simulink library "outp"  (R2021b)
(part 8 of 11)

      link override Signal_Override/_ovrdval: Value=KOUTP_FDCTHCREVentModeSta_enum_ovrdval
  VTHC_FDCTHCREVentYStaSet1_enum_Inproc : FVT_lib/outp/OverrideAndLimit  SystemSampleTime=-1  VariantActivationTime=update diagram  Latency=0  AutoFrameSizeCalculation=off
      link override Signal_Limit/_maxval: Value=KOUTP_FDCTHCREVentYStaSet1_enum_maxval
      link override Signal_Limit/_minval: Value=KOUTP_FDCTHCREVentYStaSet1_enum_minval
      link override Signal_Override/_ovrdflg: Value=KOUTP_FDCTHCREVentYStaSet1_enum_ovrdflg
      link override Signal_Override/_ovrdval: Value=KOUTP_FDCTHCREVentYStaSet1_enum_ovrdval
  VTHC_FDCTHCREVentYStaSet2_enum_Inproc : FVT_lib/outp/OverrideAndLimit  SystemSampleTime=-1  VariantActivationTime=update diagram  Latency=0  AutoFrameSizeCalculation=off
      link override Signal_Limit/_maxval: Value=KOUTP_FDCTHCREVentYStaSet2_enum_maxval
      link override Signal_Limit/_minval: Value=KOUTP_FDCTHCREVentYStaSet2_enum_minval
      link override Signal_Override/_ovrdflg: Value=KOUTP_FDCTHCREVentYStaSet2_enum_ovrdflg
      link override Signal_Override/_ovrdval: Value=KOUTP_FDCTHCREVentYStaSet2_enum_ovrdval
  VTHC_FDCTHCREVentYStaSet3_enum_Inproc : FVT_lib/outp/OverrideAndLimit  SystemSampleTime=-1  VariantActivationTime=update diagram  Latency=0  AutoFrameSizeCalculation=off
      link override Signal_Limit/_maxval: Value=KOUTP_FDCTHCREVentYStaSet3_enum_maxval
      link override Signal_Limit/_minval: Value=KOUTP_FDCTHCREVentYStaSet3_enum_minval
      link override Signal_Override/_ovrdflg: Value=KOUTP_FDCTHCREVentYStaSet3_enum_ovrdflg
      link override Signal_Override/_ovrdval: Value=KOUTP_FDCTHCREVentYStaSet3_enum_ovrdval
  VTHC_FDCTHCREVentYStaSet4_enum_Inproc : FVT_lib/outp/OverrideAndLimit  SystemSampleTime=-1  VariantActivationTime=update diagram  Latency=0  AutoFrameSizeCalculation=off
      link override Signal_Limit/_maxval: Value=KOUTP_FDCTHCREVentYStaSet4_enum_maxval
      link override Signal_Limit/_minval: Value=KOUTP_FDCTHCREVentYStaSet4_enum_minval
      link override Signal_Override/_ovrdflg: Value=KOUTP_FDCTHCREVentYStaSet4_enum_ovrdflg
      link override Signal_Override/_ovrdval: Value=KOUTP_FDCTHCREVentYStaSet4_enum_ovrdval
  VTHC_FDCTHCREVentYStaSet5_enum_Inproc : FVT_lib/outp/OverrideAndLimit  SystemSampleTime=-1  VariantActivationTime=update diagram  Latency=0  AutoFrameSizeCalculation=off
      link override Signal_Limit/_maxval: Value=KOUTP_FDCTHCREVentYStaSet5_enum_maxval
      link override Signal_Limit/_minval: Value=KOUTP_FDCTHCREVentYStaSet5_enum_minval
      link override Signal_Override/_ovrdflg: Value=KOUTP_FDCTHCREVentYStaSet5_enum_ovrdflg
      link override Signal_Override/_ovrdval: Value=KOUTP_FDCTHCREVentYStaSet5_enum_ovrdval
  VTHC_FDCTHCREVentYStaSet7_enum_Inproc : FVT_lib/outp/OverrideAndLimit  SystemSampleTime=-1  VariantActivationTime=update diagram  Latency=0  AutoFrameSizeCalculation=off
      link override Signal_Limit/_maxval: Value=KOUTP_FDCTHCREVentYStaSet7_enum_maxval
      link override Signal_Limit/_minval: Value=KOUTP_FDCTHCREVentYStaSet7_enum_minval
      link override Signal_Override/_ovrdflg: Value=KOUTP_FDCTHCREVentYStaSet7_enum_ovrdflg
      link override Signal_Override/_ovrdval: Value=KOUTP_FDCTHCREVentYStaSet7_enum_ovrdval
  VTHC_FDCTHCREVentYSta_enum_Inproc : FVT_lib/outp/OverrideAndLimit  SystemSampleTime=-1  VariantActivationTime=update diagram  Latency=0  AutoFrameSizeCalculation=off
      link override Signal_Limit/_maxval: Value=KOUTP_FDCTHCREVentYSta_enum_maxval
      link override Signal_Limit/_minval: Value=KOUTP_FDCTHCREVentYSta_enum_minval
      link override Signal_Override/_ovrdflg: Value=KOUTP_FDCTHCREVentYSta_enum_ovrdflg
      link override Signal_Override/_ovrdval: Value=KOUTP_FDCTHCREVentYSta_enum_ovrdval
  VTHC_FDCTHCREVentZStaSet1_enum_Inproc : FVT_lib/outp/OverrideAndLimit  SystemSampleTime=-1  VariantActivationTime=update diagram  Latency=0  AutoFrameSizeCalculation=off
      link override Signal_Limit/_maxval: Value=KOUTP_FDCTHCREVentZStaSet1_enum_maxval
      link override Signal_Limit/_minval: Value=KOUTP_FDCTHCREVentZStaSet1_enum_minval
      link override Signal_Override/_ovrdflg: Value=KOUTP_FDCTHCREVentZStaSet1_enum_ovrdflg
      link override Signal_Override/_ovrdval: Value=KOUTP_FDCTHCREVentZStaSet1_enum_ovrdval
  VTHC_FDCTHCREVentZStaSet2_enum_Inproc : FVT_lib/outp/OverrideAndLimit  SystemSampleTime=-1  VariantActivationTime=update diagram  Latency=0  AutoFrameSizeCalculation=off
      link override Signal_Limit/_maxval: Value=KOUTP_FDCTHCREVentZStaSet2_enum_maxval
      link override Signal_Limit/_minval: Value=KOUTP_FDCTHCREVentZStaSet2_enum_minval
      link override Signal_Override/_ovrdflg: Value=KOUTP_FDCTHCREVentZStaSet2_enum_ovrdflg
      link override Signal_Override/_ovrdval: Value=KOUTP_FDCTHCREVentZStaSet2_enum_ovrdval
  VTHC_FDCTHCREVentZStaSet3_enum_Inproc : FVT_lib/outp/OverrideAndLimit  SystemSampleTime=-1  VariantActivationTime=update diagram  Latency=0  AutoFrameSizeCalculation=off
      link override Signal_Limit/_maxval: Value=KOUTP_FDCTHCREVentZStaSet3_enum_maxval
      link override Signal_Limit/_minval: Value=KOUTP_FDCTHCREVentZStaSet3_enum_minval
      link override Signal_Override/_ovrdflg: Value=KOUTP_FDCTHCREVentZStaSet3_enum_ovrdflg
      link override Signal_Override/_ovrdval: Value=KOUTP_FDCTHCREVentZStaSet3_enum_ovrdval
  VTHC_FDCTHCREVentZStaSet4_enum_Inproc : FVT_lib/outp/OverrideAndLimit  SystemSampleTime=-1  VariantActivationTime=update diagram  Latency=0  AutoFrameSizeCalculation=off
      link override Signal_Limit/_maxval: Value=KOUTP_FDCTHCREVentZStaSet4_enum_maxval
      link override Signal_Limit/_minval: Value=KOUTP_FDCTHCREVentZStaSet4_enum_minval
      link override Signal_Override/_ovrdflg: Value=KOUTP_FDCTHCREVentZStaSet4_enum_ovrdflg
      link override Signal_Override/_ovrdval: Value=KOUTP_FDCTHCREVentZStaSet4_enum_ovrdval
  VTHC_FDCTHCREVentZStaSet5_enum_Inproc : FVT_lib/outp/OverrideAndLimit  SystemSampleTime=-1  VariantActivationTime=update diagram  Latency=0  AutoFrameSizeCalculation=off
      link override Signal_Limit/_maxval: Value=KOUTP_FDCTHCREVentZStaSet5_enum_maxval
      link override Signal_Limit/_minval: Value=KOUTP_FDCTHCREVentZStaSet5_enum_minval
      link override Signal_Override/_ovrdflg: Value=KOUTP_FDCTHCREVentZStaSet5_enum_ovrdflg
      link override Signal_Override/_ovrdval: Value=KOUTP_FDCTHCREVentZStaSet5_enum_ovrdval
  VTHC_FDCTHCREVentZStaSet7_enum_Inproc : FVT_lib/outp/OverrideAndLimit  SystemSampleTime=-1  VariantActivationTime=update diagram  Latency=0  AutoFrameSizeCalculation=off
      link override Signal_Limit/_maxval: Value=KOUTP_FDCTHCREVentZStaSet7_enum_maxval
      link override Signal_Limit/_minval: Value=KOUTP_FDCTHCREVentZStaSet7_enum_minval
      link override Signal_Override/_ovrdflg: Value=KOUTP_FDCTHCREVentZStaSet7_enum_ovrdflg
      link override Signal_Override/_ovrdval: Value=KOUTP_FDCTHCREVentZStaSet7_enum_ovrdval
  VTHC_FDCTHCREVentZSta_enum_Inproc : FVT_lib/outp/OverrideAndLimit  SystemSampleTime=-1  VariantActivationTime=update diagram  Latency=0  AutoFrameSizeCalculation=off
      link override Signal_Limit/_maxval: Value=KOUTP_FDCTHCREVentZSta_enum_maxval
      link override Signal_Limit/_minval: Value=KOUTP_FDCTHCREVentZSta_enum_minval
      link override Signal_Override/_ovrdflg: Value=KOUTP_FDCTHCREVentZSta_enum_ovrdflg
      link override Signal_Override/_ovrdval: Value=KOUTP_FDCTHCREVentZSta_enum_ovrdval
  VTHC_FDCTHCRVentENSta_flg_Inproc : FVT_lib/outp/OverrideAndLimit  SystemSampleTime=-1  VariantActivationTime=update diagram  Latency=0  AutoFrameSizeCalculation=off
      link override Signal_Limit/_maxval: Value=KOUTP_FDCTHCRVentENSta_flg_maxval
      link override Signal_Limit/_minval: Value=KOUTP_FDCTHCRVentENSta_flg_minval
      link override Signal_Override/_ovrdflg: Value=KOUTP_FDCTHCRVentENSta_flg_ovrdflg
      link override Signal_Override/_ovrdval: Value=KOUTP_FDCTHCRVentENSta_flg_ovrdval
  VTHC_FDCompCmd_rpm_Inproc : FVT_lib/outp/OverrideAndLimit  SystemSampleTime=-1  VariantActivationTime=update diagram  Latency=0  AutoFrameSizeCalculation=off
      link override Signal_Limit/_maxval: Value=KOUTP_FDCompCmd_rpm_maxval
      link override Signal_Limit/_minval: Value=KOUTP_FDCompCmd_rpm_minval
      link override Signal_Override/_ovrdflg: Value=KOUTP_FDCompCmd_rpm_ovrdflg
      link override Signal_Override/_ovrdval: Value=KOUTP_FDCompCmd_rpm_ovrdval
  VTHC_FDEWP1Cmd_enum_Inproc : FVT_lib/outp/OverrideAndLimit  SystemSampleTime=-1  VariantActivationTime=update diagram  Latency=0  AutoFrameSizeCalculation=off
      link override Signal_Limit/_maxval: Value=KOUTP_FDEWP1Cmd_enum_maxval
      link override Signal_Limit/_minval: Value=KOUTP_FDEWP1Cmd_enum_minval
      link override Signal_Override/_ovrdflg: Value=KOUTP_FDEWP1Cmd_enum_ovrdflg
      link override Signal_Override/_ovrdval: Value=KOUTP_FDEWP1Cmd_enum_ovrdval
  VTHC_FDEWP2Cmd_enum_Inproc : FVT_lib/outp/OverrideAndLimit  SystemSampleTime=-1  VariantActivationTime=update diagram  Latency=0  AutoFrameSizeCalculation=off
      link override Signal_Limit/_maxval: Value=KOUTP_FDEWP2Cmd_enum_maxval
      link override Signal_Limit/_minval: Value=KOUTP_FDEWP2Cmd_enum_minval
      link override Signal_Override/_ovrdflg: Value=KOUTP_FDEWP2Cmd_enum_ovrdflg
      link override Signal_Override/_ovrdval: Value=KOUTP_FDEWP2Cmd_enum_ovrdval
  VTHC_FDEWP3Cmd_enum_Inproc : FVT_lib/outp/OverrideAndLimit  SystemSampleTime=-1  VariantActivationTime=update diagram  Latency=0  AutoFrameSizeCalculation=off
      link override Signal_Limit/_maxval: Value=KOUTP_FDEWP3Cmd_enum_maxval
      link override Signal_Limit/_minval: Value=KOUTP_FDEWP3Cmd_enum_minval
      link override Signal_Override/_ovrdflg: Value=KOUTP_FDEWP3Cmd_enum_ovrdflg
      link override Signal_Override/_ovrdval: Value=KOUTP_FDEWP3Cmd_enum_ovrdval
  VTHC_FDEXV1Cmd_step_Inproc : FVT_lib/outp/OverrideAndLimit  SystemSampleTime=-1  VariantActivationTime=update diagram  Latency=0  AutoFrameSizeCalculation=off
      link override Signal_Limit/_maxval: Value=KOUTP_FDEXV1Cmd_step_maxval
      link override Signal_Limit/_minval: Value=KOUTP_FDEXV1Cmd_step_minval
      link override Signal_Override/_ovrdflg: Value=KOUTP_FDEXV1Cmd_step_ovrdflg
      link override Signal_Override/_ovrdval: Value=KOUTP_FDEXV1Cmd_step_ovrdval
  VTHC_FDEXV2Cmd_step_Inproc : FVT_lib/outp/OverrideAndLimit  SystemSampleTime=-1  VariantActivationTime=update diagram  Latency=0  AutoFrameSizeCalculation=off
      link override Signal_Limit/_maxval: Value=KOUTP_FDEXV2Cmd_step_maxval
      link override Signal_Limit/_minval: Value=KOUTP_FDEXV2Cmd_step_minval
      link override Signal_Override/_ovrdflg: Value=KOUTP_FDEXV2Cmd_step_ovrdflg
      link override Signal_Override/_ovrdval: Value=KOUTP_FDEXV2Cmd_step_ovrdval
  VTHC_FDFWVCmd_flg_Inproc : FVT_lib/outp/OverrideAndLimit  SystemSampleTime=-1  VariantActivationTime=update diagram  Latency=0  AutoFrameSizeCalculation=off
      link override Signal_Limit/_maxval: Value=KOUTP_FDFWVCmd_flg_maxval
      link override Signal_Limit/_minval: Value=KOUTP_FDFWVCmd_flg_minval
      link override Signal_Override/_ovrdflg: Value=KOUTP_FDFWVCmd_flg_ovrdflg
      link override Signal_Override/_ovrdval: Value=KOUTP_FDFWVCmd_flg_ovrdval
  VTHC_FDFrLeAPTCHeatPwrCmd_W_Inproc : FVT_lib/outp/OverrideAndLimit  SystemSampleTime=-1  VariantActivationTime=update diagram  Latency=0  AutoFrameSizeCalculation=off
      link override Signal_Limit/_maxval: Value=KOUTP_FDFrLeAPTCHeatPwrCmd_W_maxval
      link override Signal_Limit/_minval: Value=KOUTP_FDFrLeAPTCHeatPwrCmd_W_minval
      link override Signal_Override/_ovrdflg: Value=KOUTP_FDFrLeAPTCHeatPwrCmd_W_ovrdflg
      link override Signal_Override/_ovrdval: Value=KOUTP_FDFrLeAPTCHeatPwrCmd_W_ovrdval
  VTHC_FDFrRiAPTCHeatPwrCmd_W_Inproc : FVT_lib/outp/OverrideAndLimit  SystemSampleTime=-1  VariantActivationTime=update diagram  Latency=0  AutoFrameSizeCalculation=off
      link override Signal_Limit/_maxval: Value=KOUTP_FDFrRiAPTCHeatPwrCmd_W_maxval
      link override Signal_Limit/_minval: Value=KOUTP_FDFrRiAPTCHeatPwrCmd_W_minval
      link override Signal_Override/_ovrdflg: Value=KOUTP_FDFrRiAPTCHeatPwrCmd_W_ovrdflg
      link override Signal_Override/_ovrdval: Value=KOUTP_FDFrRiAPTCHeatPwrCmd_W_ovrdval
  VTHC_FDFrWPTCHeatPwrCmd_W_Inproc : FVT_lib/outp/OverrideAndLimit  SystemSampleTime=-1  VariantActivationTime=update diagram  Latency=0  AutoFrameSizeCalculation=off
      link override Signal_Limit/_maxval: Value=KOUTP_FDFrWPTCHeatPwrCmd_W_maxval
      link override Signal_Limit/_minval: Value=KOUTP_FDFrWPTCHeatPwrCmd_W_minval
      link override Signal_Override/_ovrdflg: Value=KOUTP_FDFrWPTCHeatPwrCmd_W_ovrdflg
      link override Signal_Override/_ovrdval: Value=KOUTP_FDFrWPTCHeatPwrCmd_W_ovrdval
  VTHC_FDRecyAutoCmd_enum_Inproc : FVT_lib/outp/OverrideAndLimit  SystemSampleTime=-1  VariantActivationTime=update diagram  Latency=0  AutoFrameSizeCalculation=off
      link override Signal_Limit/_maxval: Value=KOUTP_FDRecyAutoCmd_enum_maxval
      link override Signal_Limit/_minval: Value=KOUTP_FDRecyAutoCmd_enum_minval
      link override Signal_Override/_ovrdflg: Value=KOUTP_FDRecyAutoCmd_enum_ovrdflg
      link override Signal_Override/_ovrdval: Value=KOUTP_FDRecyAutoCmd_enum_ovrdval
  VTHC_FDRrAPTCHeatPwrCmd_W_Inproc : FVT_lib/outp/OverrideAndLimit  SystemSampleTime=-1  VariantActivationTime=update diagram  Latency=0  AutoFrameSizeCalculation=off
      link override Signal_Limit/_maxval: Value=KOUTP_FDRrAPTCHeatPwrCmd_W_maxval
      link override Signal_Limit/_minval: Value=KOUTP_FDRrAPTCHeatPwrCmd_W_minval
      link override Signal_Override/_ovrdflg: Value=KOUTP_FDRrAPTCHeatPwrCmd_W_ovrdflg
      link override Signal_Override/_ovrdval: Value=KOUTP_FDRrAPTCHeatPwrCmd_W_ovrdval
  VTHC_FDSOTXVCmd_flg_Inproc : FVT_lib/outp/OverrideAndLimit  SystemSampleTime=-1  VariantActivationTime=update diagram  Latency=0  AutoFrameSizeCalculation=off
      link override Signal_Limit/_maxval: Value=KOUTP_FDSOTXVCmd_flg_maxval
      link override Signal_Limit/_minval: Value=KOUTP_FDSOTXVCmd_flg_minval
      link override Signal_Override/_ovrdflg: Value=KOUTP_FDSOTXVCmd_flg_ovrdflg
      link override Signal_Override/_ovrdval: Value=KOUTP_FDSOTXVCmd_flg_ovrdval
  VTHC_FDSOV1Cmd_flg_Inproc : FVT_lib/outp/OverrideAndLimit  SystemSampleTime=-1  VariantActivationTime=update diagram  Latency=0  AutoFrameSizeCalculation=off
      link override Signal_Limit/_maxval: Value=KOUTP_FDSOV1Cmd_flg_maxval
      link override Signal_Limit/_minval: Value=KOUTP_FDSOV1Cmd_flg_minval
      link override Signal_Override/_ovrdflg: Value=KOUTP_FDSOV1Cmd_flg_ovrdflg
      link override Signal_Override/_ovrdval: Value=KOUTP_FDSOV1Cmd_flg_ovrdval
  VTHC_FDSOV2Cmd_flg_Inproc : FVT_lib/outp/OverrideAndLimit  SystemSampleTime=-1  VariantActivationTime=update diagram  Latency=0  AutoFrameSizeCalculation=off
      link override Signal_Limit/_maxval: Value=KOUTP_FDSOV2Cmd_flg_maxval
      link override Signal_Limit/_minval: Value=KOUTP_FDSOV2Cmd_flg_minval
      link override Signal_Override/_ovrdflg: Value=KOUTP_FDSOV2Cmd_flg_ovrdflg
      link override Signal_Override/_ovrdval: Value=KOUTP_FDSOV2Cmd_flg_ovrdval
  VTHC_FDSOV3Cmd_flg_Inproc : FVT_lib/outp/OverrideAndLimit  SystemSampleTime=-1  VariantActivationTime=update diagram  Latency=0  AutoFrameSizeCalculation=off
      link override Signal_Limit/_maxval: Value=KOUTP_FDSOV3Cmd_flg_maxval
      link override Signal_Limit/_minval: Value=KOUTP_FDSOV3Cmd_flg_minval
      link override Signal_Override/_ovrdflg: Value=KOUTP_FDSOV3Cmd_flg_ovrdflg
      link override Signal_Override/_ovrdval: Value=KOUTP_FDSOV3Cmd_flg_ovrdval
  VTHC_FDTWVCmd_pct_Inproc : FVT_lib/outp/OverrideAndLimit  SystemSampleTime=-1  VariantActivationTime=update diagram  Latency=0  AutoFrameSizeCalculation=off
      link override Signal_Limit/_maxval: Value=KOUTP_FDTWVCmd_pct_maxval
      link override Signal_Limit/_minval: Value=KOUTP_FDTWVCmd_pct_minval
      link override Signal_Override/_ovrdflg: Value=KOUTP_FDTWVCmd_pct_ovrdflg
      link override Signal_Override/_ovrdval: Value=KOUTP_FDTWVCmd_pct_ovrdval
  VTHC_FOOTSet_enum_Inproc : FVT_lib/outp/OverrideAndLimit  SystemSampleTime=-1  VariantActivationTime=update diagram  Latency=0  AutoFrameSizeCalculation=off
      link override Signal_Limit/_maxval: Value=KOUTP_FOOTSet_enum_maxval
      link override Signal_Limit/_minval: Value=KOUTP_FOOTSet_enum_minval
      link override Signal_Override/_ovrdflg: Value=KOUTP_FOOTSet_enum_ovrdflg
      link override Signal_Override/_ovrdval: Value=KOUTP_FOOTSet_enum_ovrdval
  VTHC_FaceMSet_enum_Inproc : FVT_lib/outp/OverrideAndLimit  SystemSampleTime=-1  VariantActivationTime=update diagram  Latency=0  AutoFrameSizeCalculation=off
      link override Signal_Limit/_maxval: Value=KOUTP_FaceMSet_enum_maxval
      link override Signal_Limit/_minval: Value=KOUTP_FaceMSet_enum_minval
      link override Signal_Override/_ovrdflg: Value=KOUTP_FaceMSet_enum_ovrdflg
      link override Signal_Override/_ovrdval: Value=KOUTP_FaceMSet_enum_ovrdval
  VTHC_FaceM_flg_Inproc : FVT_lib/outp/OverrideAndLimit  SystemSampleTime=-1  VariantActivationTime=update diagram  Latency=0  AutoFrameSizeCalculation=off
      link override Signal_Limit/_maxval: Value=KOUTP_FaceM_flg_maxval
      link override Signal_Limit/_minval: Value=KOUTP_FaceM_flg_minval
      link override Signal_Override/_ovrdflg: Value=KOUTP_FaceM_flg_ovrdflg
      link override Signal_Override/_ovrdval: Value=KOUTP_FaceM_flg_ovrdval
  VTHC_Face_flg_Inproc : FVT_lib/outp/OverrideAndLimit  SystemSampleTime=-1  VariantActivationTime=update diagram  Latency=0  AutoFrameSizeCalculation=off
      link override Signal_Limit/_maxval: Value=KOUTP_Face_flg_maxval
      link override Signal_Limit/_minval: Value=KOUTP_Face_flg_minval
      link override Signal_Override/_ovrdflg: Value=KOUTP_Face_flg_ovrdflg
      link override Signal_Override/_ovrdval: Value=KOUTP_Face_flg_ovrdval
  VTHC_FootMSet_enum_Inproc : FVT_lib/outp/OverrideAndLimit  SystemSampleTime=-1  VariantActivationTime=update diagram  Latency=0  AutoFrameSizeCalculation=off
      link override Signal_Limit/_maxval: Value=KOUTP_FootMSet_enum_maxval
      link override Signal_Limit/_minval: Value=KOUTP_FootMSet_enum_minval
      link override Signal_Override/_ovrdflg: Value=KOUTP_FootMSet_enum_ovrdflg
      link override Signal_Override/_ovrdval: Value=KOUTP_FootMSet_enum_ovrdval
  VTHC_FootM_flg_Inproc : FVT_lib/outp/OverrideAndLimit  SystemSampleTime=-1  VariantActivationTime=update diagram  Latency=0  AutoFrameSizeCalculation=off
      link override Signal_Limit/_maxval: Value=KOUTP_FootM_flg_maxval
      link override Signal_Limit/_minval: Value=KOUTP_FootM_flg_minval
      link override Signal_Override/_ovrdflg: Value=KOUTP_FootM_flg_ovrdflg
      link override Signal_Override/_ovrdval: Value=KOUTP_FootM_flg_ovrdval
  VTHC_Foot_flg_Inproc : FVT_lib/outp/OverrideAndLimit  SystemSampleTime=-1  VariantActivationTime=update diagram  Latency=0  AutoFrameSizeCalculation=off
      link override Signal_Limit/_maxval: Value=KOUTP_Foot_flg_maxval
      link override Signal_Limit/_minval: Value=KOUTP_Foot_flg_minval
      link override Signal_Override/_ovrdflg: Value=KOUTP_Foot_flg_ovrdflg
      link override Signal_Override/_ovrdval: Value=KOUTP_Foot_flg_ovrdval
  VTHC_FrostSet_enum_Inproc : FVT_lib/outp/OverrideAndLimit  SystemSampleTime=-1  VariantActivationTime=update diagram  Latency=0  AutoFrameSizeCalculation=off
      link override Signal_Limit/_maxval: Value=KOUTP_FrostSet_enum_maxval
      link override Signal_Limit/_minval: Value=KOUTP_FrostSet_enum_minval
      link override Signal_Override/_ovrdflg: Value=KOUTP_FrostSet_enum_ovrdflg
      link override Signal_Override/_ovrdval: Value=KOUTP_FrostSet_enum_ovrdval
  VTHC_Frost_flg_Inproc : FVT_lib/outp/OverrideAndLimit  SystemSampleTime=-1  VariantActivationTime=update diagram  Latency=0  AutoFrameSizeCalculation=off
      link override Signal_Limit/_maxval: Value=KOUTP_Frost_flg_maxval
      link override Signal_Limit/_minval: Value=KOUTP_Frost_flg_minval
      link override Signal_Override/_ovrdflg: Value=KOUTP_Frost_flg_ovrdflg
      link override Signal_Override/_ovrdval: Value=KOUTP_Frost_flg_ovrdval
  VTHC_IONSWStaSet_enum_Inproc : FVT_lib/outp/OverrideAndLimit  SystemSampleTime=-1  VariantActivationTime=update diagram  Latency=0  AutoFrameSizeCalculation=off
      link override Signal_Limit/_maxval: Value=KOUTP_IONSWStaSet_enum_maxval
      link override Signal_Limit/_minval: Value=KOUTP_IONSWStaSet_enum_minval
      link override Signal_Override/_ovrdflg: Value=KOUTP_IONSWStaSet_enum_ovrdflg
      link override Signal_Override/_ovrdval: Value=KOUTP_IONSWStaSet_enum_ovrdval
  VTHC_LEVentModeStaSet123_enum_Inproc : FVT_lib/outp/OverrideAndLimit  SystemSampleTime=-1  VariantActivationTime=update diagram  Latency=0  AutoFrameSizeCalculation=off
      link override Signal_Limit/_maxval: Value=KOUTP_LEVentModeStaSet123_enum_maxval
      link override Signal_Limit/_minval: Value=KOUTP_LEVentModeStaSet123_enum_minval
      link override Signal_Override/_ovrdflg: Value=KOUTP_LEVentModeStaSet123_enum_ovrdflg
      link override Signal_Override/_ovrdval: Value=KOUTP_LEVentModeStaSet123_enum_ovrdval
  VTHC_LEVentModeStaSet457_enum_Inproc : FVT_lib/outp/OverrideAndLimit  SystemSampleTime=-1  VariantActivationTime=update diagram  Latency=0  AutoFrameSizeCalculation=off
      link override Signal_Limit/_maxval: Value=KOUTP_LEVentModeStaSet457_enum_maxval
      link override Signal_Limit/_minval: Value=KOUTP_LEVentModeStaSet457_enum_minval
      link override Signal_Override/_ovrdflg: Value=KOUTP_LEVentModeStaSet457_enum_ovrdflg
      link override Signal_Override/_ovrdval: Value=KOUTP_LEVentModeStaSet457_enum_ovrdval
  VTHC_LVentENSet_enum_Inproc : FVT_lib/outp/OverrideAndLimit  SystemSampleTime=-1  VariantActivationTime=update diagram  Latency=0  AutoFrameSizeCalculation=off
      link override Signal_Limit/_maxval: Value=KOUTP_LVentENSet_enum_maxval
      link override Signal_Limit/_minval: Value=KOUTP_LVentENSet_enum_minval
      link override Signal_Override/_ovrdflg: Value=KOUTP_LVentENSet_enum_ovrdflg
      link override Signal_Override/_ovrdval: Value=KOUTP_LVentENSet_enum_ovrdval
  VTHC_LVentEN_flg_Inproc : FVT_lib/outp/OverrideAndLimit  SystemSampleTime=-1  VariantActivationTime=update diagram  Latency=0  AutoFrameSizeCalculation=off
      link override Signal_Limit/_maxval: Value=KOUTP_LVentEN_flg_maxval
      link override Signal_Limit/_minval: Value=KOUTP_LVentEN_flg_minval
      link override Signal_Override/_ovrdflg: Value=KOUTP_LVentEN_flg_ovrdflg
      link override Signal_Override/_ovrdval: Value=KOUTP_LVentEN_flg_ovrdval
  VTHC_REVentModeStaSet123_enum_Inproc : FVT_lib/outp/OverrideAndLimit  SystemSampleTime=-1  VariantActivationTime=update diagram  Latency=0  AutoFrameSizeCalculation=off
      link override Signal_Limit/_maxval: Value=KOUTP_REVentModeStaSet123_enum_maxval
      link override Signal_Limit/_minval: Value=KOUTP_REVentModeStaSet123_enum_minval
      link override Signal_Override/_ovrdflg: Value=KOUTP_REVentModeStaSet123_enum_ovrdflg
      link override Signal_Override/_ovrdval: Value=KOUTP_REVentModeStaSet123_enum_ovrdval
  VTHC_REVentModeStaSet457_enum_Inproc : FVT_lib/outp/OverrideAndLimit  SystemSampleTime=-1  VariantActivationTime=update diagram  Latency=0  AutoFrameSizeCalculation=off
      link override Signal_Limit/_maxval: Value=KOUTP_REVentModeStaSet457_enum_maxval
      link override Signal_Limit/_minval: Value=KOUTP_REVentModeStaSet457_enum_minval
      link override Signal_Override/_ovrdflg: Value=KOUTP_REVentModeStaSet457_enum_ovrdflg
      link override Signal_Override/_ovrdval: Value=KOUTP_REVentModeStaSet457_enum_ovrdval
  VTHC_RVentENSet_enum_Inproc : FVT_lib/outp/OverrideAndLimit  SystemSampleTime=-1  VariantActivationTime=update diagram  Latency=0  AutoFrameSizeCalculation=off
      link override Signal_Limit/_maxval: Value=KOUTP_RVentENSet_enum_maxval
      link override Signal_Limit/_minval: Value=KOUTP_RVentENSet_enum_minval
      link override Signal_Override/_ovrdflg: Value=KOUTP_RVentENSet_enum_ovrdflg
      link override Signal_Override/_ovrdval: Value=KOUTP_RVentENSet_enum_ovrdval
  VTHC_RVentEN_flg_Inproc : FVT_lib/outp/OverrideAndLimit  SystemSampleTime=-1  VariantActivationTime=update diagram  Latency=0  AutoFrameSizeCalculation=off
      link override Signal_Limit/_maxval: Value=KOUTP_RVentEN_flg_maxval
      link override Signal_Limit/_minval: Value=KOUTP_RVentEN_flg_minval
      link override Signal_Override/_ovrdflg: Value=KOUTP_RVentEN_flg_ovrdflg
      link override Signal_Override/_ovrdval: Value=KOUTP_RVentEN_flg_ovrdval
  VTHC_RecAutoFlg_flg_Inproc : FVT_lib/outp/OverrideAndLimit  SystemSampleTime=-1  VariantActivationTime=update diagram  Latency=0  AutoFrameSizeCalculation=off
      link override Signal_Limit/_maxval: Value=KOUTP_RecAutoFlg_flg_maxval
      link override Signal_Limit/_minval: Value=KOUTP_RecAutoFlg_flg_minval
      link override Signal_Override/_ovrdflg: Value=KOUTP_RecAutoFlg_flg_ovrdflg
      link override Signal_Override/_ovrdval: Value=KOUTP_RecAutoFlg_flg_ovrdval
  VTHC_RecyAutoSet_enum_Inproc : FVT_lib/outp/OverrideAndLimit  SystemSampleTime=-1  VariantActivationTime=update diagram  Latency=0  AutoFrameSizeCalculation=off
      link override Signal_Limit/_maxval: Value=KOUTP_RecyAutoSet_enum_maxval
      link override Signal_Limit/_minval: Value=KOUTP_RecyAutoSet_enum_minval
      link override Signal_Override/_ovrdflg: Value=KOUTP_RecyAutoSet_enum_ovrdflg
      link override Signal_Override/_ovrdval: Value=KOUTP_RecyAutoSet_enum_ovrdval
  VTHC_SettempZon1Set1_enum_Inproc : FVT_lib/outp/OverrideAndLimit  SystemSampleTime=-1  VariantActivationTime=update diagram  Latency=0  AutoFrameSizeCalculation=off
      link override Signal_Limit/_maxval: Value=KOUTP_SettempZon1Set1_enum_maxval
      link override Signal_Limit/_minval: Value=KOUTP_SettempZon1Set1_enum_minval
      link override Signal_Override/_ovrdflg: Value=KOUTP_SettempZon1Set1_enum_ovrdflg
      link override Signal_Override/_ovrdval: Value=KOUTP_SettempZon1Set1_enum_ovrdval
  VTHC_SettempZon1Set2_enum_Inproc : FVT_lib/outp/OverrideAndLimit  SystemSampleTime=-1  VariantActivationTime=update diagram  Latency=0  AutoFrameSizeCalculation=off
      link override Signal_Limit/_maxval: Value=KOUTP_SettempZon1Set2_enum_maxval
      link override Signal_Limit/_minval: Value=KOUTP_SettempZon1Set2_enum_minval
      link override Signal_Override/_ovrdflg: Value=KOUTP_SettempZon1Set2_enum_ovrdflg
      link override Signal_Override/_ovrdval: Value=KOUTP_SettempZon1Set2_enum_ovrdval
  VTHC_SettempZon1Set3_enum_Inproc : FVT_lib/outp/OverrideAndLimit  SystemSampleTime=-1  VariantActivationTime=update diagram  Latency=0  AutoFrameSizeCalculation=off
      link override Signal_Limit/_maxval: Value=KOUTP_SettempZon1Set3_enum_maxval
      link override Signal_Limit/_minval: Value=KOUTP_SettempZon1Set3_enum_minval
      link override Signal_Override/_ovrdflg: Value=KOUTP_SettempZon1Set3_enum_ovrdflg
      link override Signal_Override/_ovrdval: Value=KOUTP_SettempZon1Set3_enum_ovrdval
  VTHC_SettempZon1Set4_enum_Inproc : FVT_lib/outp/OverrideAndLimit  SystemSampleTime=-1  VariantActivationTime=update diagram  Latency=0  AutoFrameSizeCalculation=off
      link override Signal_Limit/_maxval: Value=KOUTP_SettempZon1Set4_enum_maxval
      link override Signal_Limit/_minval: Value=KOUTP_SettempZon1Set4_enum_minval
      link override Signal_Override/_ovrdflg: Value=KOUTP_SettempZon1Set4_enum_ovrdflg
      link override Signal_Override/_ovrdval: Value=KOUTP_SettempZon1Set4_enum_ovrdval
  VTHC_SettempZon1Set5_enum_Inproc : FVT_lib/outp/OverrideAndLimit  SystemSampleTime=-1  VariantActivationTime=update diagram  Latency=0  AutoFrameSizeCalculation=off
      link override Signal_Limit/_maxval: Value=KOUTP_SettempZon1Set5_enum_maxval
      link override Signal_Limit/_minval: Value=KOUTP_SettempZon1Set5_enum_minval
      link override Signal_Override/_ovrdflg: Value=KOUTP_SettempZon1Set5_enum_ovrdflg
      link override Signal_Override/_ovrdval: Value=KOUTP_SettempZon1Set5_enum_ovrdval
  VTHC_SettempZon1Set7_enum_Inproc : FVT_lib/outp/OverrideAndLimit  SystemSampleTime=-1  VariantActivationTime=update diagram  Latency=0  AutoFrameSizeCalculation=off
      link override Signal_Limit/_maxval: Value=KOUTP_SettempZon1Set7_enum_maxval
      link override Signal_Limit/_minval: Value=KOUTP_SettempZon1Set7_enum_minval
      link override Signal_Override/_ovrdflg: Value=KOUTP_SettempZon1Set7_enum_ovrdflg
      link override Signal_Override/_ovrdval: Value=KOUTP_SettempZon1Set7_enum_ovrdval
  VTHC_THSysErrlampReq_flg_Inproc : FVT_lib/outp/OverrideAndLimit  SystemSampleTime=-1  VariantActivationTime=update diagram  Latency=0  AutoFrameSizeCalculation=off
      link override Signal_Limit/_maxval: Value=KOUTP_THSysErrlampReq_flg_maxval
      link override Signal_Limit/_minval: Value=KOUTP_THSysErrlampReq_flg_minval
      link override Signal_Override/_ovrdflg: Value=KOUTP_THSysErrlampReq_flg_ovrdflg
      link override Signal_Override/_ovrdval: Value=KOUTP_THSysErrlampReq_flg_ovrdval
  VTHC_fdefogSet_enum_Inproc : FVT_lib/outp/OverrideAndLimit  SystemSampleTime=-1  VariantActivationTime=update diagram  Latency=0  AutoFrameSizeCalculation=off
      link override Signal_Limit/_maxval: Value=KOUTP_fdefogSet_enum_maxval
      link override Signal_Limit/_minval: Value=KOUTP_fdefogSet_enum_minval
      link override Signal_Override/_ovrdflg: Value=KOUTP_fdefogSet_enum_ovrdflg
      link override Signal_Override/_ovrdval: Value=KOUTP_fdefogSet_enum_ovrdval
  VTHC_fdefog_flg_Inproc : FVT_lib/outp/OverrideAndLimit  SystemSampleTime=-1  VariantActivationTime=update diagram  Latency=0  AutoFrameSizeCalculation=off
      link override Signal_Limit/_maxval: Value=KOUTP_fdefog_flg_maxval
      link override Signal_Limit/_minval: Value=KOUTP_fdefog_flg_minval
      link override Signal_Override/_ovrdflg: Value=KOUTP_fdefog_flg_ovrdflg
      link override Signal_Override/_ovrdval: Value=KOUTP_fdefog_flg_ovrdval
  VTHC_sigAirIntenZon1St_enum_Inproc : FVT_lib/outp/OverrideAndLimit  SystemSampleTime=-1  VariantActivationTime=update diagram  Latency=0  AutoFrameSizeCalculation=off
      link override Signal_Limit/_maxval: Value=KOUTP_sigAirIntenZon1St_enum_maxval
      link override Signal_Limit/_minval: Value=KOUTP_sigAirIntenZon1St_enum_minval
      link override Signal_Override/_ovrdflg: Value=KOUTP_sigAirIntenZon1St_enum_ovrdflg
      link override Signal_Override/_ovrdval: Value=KOUTP_sigAirIntenZon1St_enum_ovrdval
  VTHC_sigAmbAirT_C_Inproc : FVT_lib/outp/OverrideAndLimit  SystemSampleTime=-1  VariantActivationTime=update diagram  Latency=0  AutoFrameSizeCalculation=off
      link override Signal_Limit/_maxval: Value=KOUTP_sigAmbAirT_C_maxval
      link override Signal_Limit/_minval: Value=KOUTP_sigAmbAirT_C_minval
      link override Signal_Override/_ovrdflg: Value=KOUTP_sigAmbAirT_C_ovrdflg
      link override Signal_Override/_ovrdval: Value=KOUTP_sigAmbAirT_C_ovrdval
  VTHC_sigCbnAirT_C_Inproc : FVT_lib/outp/OverrideAndLimit  SystemSampleTime=-1  VariantActivationTime=update diagram  Latency=0  AutoFrameSizeCalculation=off
      link override Signal_Limit/_maxval: Value=KOUTP_sigCbnAirT_C_maxval
      link override Signal_Limit/_minval: Value=KOUTP_sigCbnAirT_C_minval
      link override Signal_Override/_ovrdflg: Value=KOUTP_sigCbnAirT_C_ovrdflg
      link override Signal_Override/_ovrdval: Value=KOUTP_sigCbnAirT_C_ovrdval
  VTHC_sigCbnPTCPwrAct_W_Inproc : FVT_lib/outp/OverrideAndLimit  SystemSampleTime=-1  VariantActivationTime=update diagram  Latency=0  AutoFrameSizeCalculation=off
      link override Signal_Limit/_maxval: Value=KOUTP_sigCbnPTCPwrAct_W_maxval
      link override Signal_Limit/_minval: Value=KOUTP_sigCbnPTCPwrAct_W_minval
      link override Signal_Override/_ovrdflg: Value=KOUTP_sigCbnPTCPwrAct_W_ovrdflg
      link override Signal_Override/_ovrdval: Value=KOUTP_sigCbnPTCPwrAct_W_ovrdval
  VTHC_sigCbnSolarLeft_W_Inproc : FVT_lib/outp/OverrideAndLimit  SystemSampleTime=-1  VariantActivationTime=update diagram  Latency=0  AutoFrameSizeCalculation=off
      link override Signal_Limit/_maxval: Value=KOUTP_sigCbnSolarLeft_W_maxval
      link override Signal_Limit/_minval: Value=KOUTP_sigCbnSolarLeft_W_minval
      link override Signal_Override/_ovrdflg: Value=KOUTP_sigCbnSolarLeft_W_ovrdflg
      link override Signal_Override/_ovrdval: Value=KOUTP_sigCbnSolarLeft_W_ovrdval
  VTHC_sigCbnSolarRight_W_Inproc : FVT_lib/outp/OverrideAndLimit  SystemSampleTime=-1  VariantActivationTime=update diagram  Latency=0  AutoFrameSizeCalculation=off
      link override Signal_Limit/_maxval: Value=KOUTP_sigCbnSolarRight_W_maxval
      link override Signal_Limit/_minval: Value=KOUTP_sigCbnSolarRight_W_minval
      link override Signal_Override/_ovrdflg: Value=KOUTP_sigCbnSolarRight_W_ovrdflg
      link override Signal_Override/_ovrdval: Value=KOUTP_sigCbnSolarRight_W_ovrdval
  VTHC_sigClntTHvBattIn_C_Inproc : FVT_lib/outp/OverrideAndLimit  SystemSampleTime=-1  VariantActivationTime=update diagram  Latency=0  AutoFrameSizeCalculation=off
      link override Signal_Limit/_maxval: Value=KOUTP_sigClntTHvBattIn_C_maxval
      link override Signal_Limit/_minval: Value=KOUTP_sigClntTHvBattIn_C_minval
      link override Signal_Override/_ovrdflg: Value=KOUTP_sigClntTHvBattIn_C_ovrdflg
      link override Signal_Override/_ovrdval: Value=KOUTP_sigClntTHvBattIn_C_ovrdval
  VTHC_sigClntTHvBattOut_C_Inproc : FVT_lib/outp/OverrideAndLimit  SystemSampleTime=-1  VariantActivationTime=update diagram  Latency=0  AutoFrameSizeCalculation=off
      link override Signal_Limit/_maxval: Value=KOUTP_sigClntTHvBattOut_C_maxval
      link override Signal_Limit/_minval: Value=KOUTP_sigClntTHvBattOut_C_minval
      link override Signal_Override/_ovrdflg: Value=KOUTP_sigClntTHvBattOut_C_ovrdflg
      link override Signal_Override/_ovrdval: Value=KOUTP_sigClntTHvBattOut_C_ovrdval
  VTHC_sigDfrstSt_flg_Inproc : FVT_lib/outp/OverrideAndLimit  SystemSampleTime=-1  VariantActivationTime=update diagram  Latency=0  AutoFrameSizeCalculation=off
      link override Signal_Limit/_maxval: Value=KOUTP_sigDfrstSt_flg_maxval
      link override Signal_Limit/_minval: Value=KOUTP_sigDfrstSt_flg_minval
      link override Signal_Override/_ovrdflg: Value=KOUTP_sigDfrstSt_flg_ovrdflg
      link override Signal_Override/_ovrdval: Value=KOUTP_sigDfrstSt_flg_ovrdval
  VTHC_sigRecircStSet_enum_Inproc : FVT_lib/outp/OverrideAndLimit  SystemSampleTime=-1  VariantActivationTime=update diagram  Latency=0  AutoFrameSizeCalculation=off
      link override Signal_Limit/_maxval: Value=KOUTP_sigRecircStSet_enum_maxval
      link override Signal_Limit/_minval: Value=KOUTP_sigRecircStSet_enum_minval
      link override Signal_Override/_ovrdflg: Value=KOUTP_sigRecircStSet_enum_ovrdflg
      link override Signal_Override/_ovrdval: Value=KOUTP_sigRecircStSet_enum_ovrdval
  VTHC_sigRecircSt_flg_Inproc : FVT_lib/outp/OverrideAndLimit  SystemSampleTime=-1  VariantActivationTime=update diagram  Latency=0  AutoFrameSizeCalculation=off
      link override Signal_Limit/_maxval: Value=KOUTP_sigRecircSt_flg_maxval
      link override Signal_Limit/_minval: Value=KOUTP_sigRecircSt_flg_minval
      link override Signal_Override/_ovrdflg: Value=KOUTP_sigRecircSt_flg_ovrdflg
      link override Signal_Override/_ovrdval: Value=KOUTP_sigRecircSt_flg_ovrdval
  VTHC_sigSetTempZon1St_C_Inproc : FVT_lib/outp/OverrideAndLimit  SystemSampleTime=-1  VariantActivationTime=update diagram  Latency=0  AutoFrameSizeCalculation=off
      link override Signal_Limit/_maxval: Value=KOUTP_sigSetTempZon1St_C_maxval
      link override Signal_Limit/_minval: Value=KOUTP_sigSetTempZon1St_C_minval
      link override Signal_Override/_ovrdflg: Value=KOUTP_sigSetTempZon1St_C_ovrdflg
      link override Signal_Override/_ovrdval: Value=KOUTP_sigSetTempZon1St_C_ovrdval
  VTHC_sigSetTempZon2StM_C_Inproc : FVT_lib/outp/OverrideAndLimit  SystemSampleTime=-1  VariantActivationTime=update diagram  Latency=0  AutoFrameSizeCalculation=off
      link override Signal_Limit/_maxval: Value=KOUTP_sigSetTempZon2StM_C_maxval
      link override Signal_Limit/_minval: Value=KOUTP_sigSetTempZon2StM_C_minval
      link override Signal_Override/_ovrdflg: Value=KOUTP_sigSetTempZon2StM_C_ovrdflg
      link override Signal_Override/_ovrdval: Value=KOUTP_sigSetTempZon2StM_C_ovrdval
  VTHC_sigSetTempZon2St_C_Inproc : FVT_lib/outp/OverrideAndLimit  SystemSampleTime=-1  VariantActivationTime=update diagram  Latency=0  AutoFrameSizeCalculation=off
      link override Signal_Limit/_maxval: Value=KOUTP_sigSetTempZon2St_C_maxval
      link override Signal_Limit/_minval: Value=KOUTP_sigSetTempZon2St_C_minval
      link override Signal_Override/_ovrdflg: Value=KOUTP_sigSetTempZon2St_C_ovrdflg
      link override Signal_Override/_ovrdval: Value=KOUTP_sigSetTempZon2St_C_ovrdval
  VTHC_sigWindDirZon1St_enum_Inproc : FVT_lib/outp/OverrideAndLimit  SystemSampleTime=-1  VariantActivationTime=update diagram  Latency=0  AutoFrameSizeCalculation=off
      link override Signal_Limit/_maxval: Value=KOUTP_sigWindDirZon1St_enum_maxval
      link override Signal_Limit/_minval: Value=KOUTP_sigWindDirZon1St_enum_minval
      link override Signal_Override/_ovrdflg: Value=KOUTP_sigWindDirZon1St_enum_ovrdflg
      link override Signal_Override/_ovrdval: Value=KOUTP_sigWindDirZon1St_enum_ovrdval
  VTPM_ALFin_flg_Inproc : FVT_lib/outp/OverrideAndLimit  SystemSampleTime=-1  VariantActivationTime=update diagram  Latency=0  AutoFrameSizeCalculation=off
      link override Signal_Limit/_maxval: Value=KOUTP_ALFin_flg_maxval
      link override Signal_Limit/_minval: Value=KOUTP_ALFin_flg_minval
      link override Signal_Override/_ovrdflg: Value=KOUTP_ALFin_flg_ovrdflg
      link override Signal_Override/_ovrdval: Value=KOUTP_ALFin_flg_ovrdval
  VTPM_AutoLTips_enum_Inproc : FVT_lib/outp/OverrideAndLimit  SystemSampleTime=-1  VariantActivationTime=update diagram  Latency=0  AutoFrameSizeCalculation=off
      link override Signal_Limit/_maxval: Value=KOUTP_AutoLTips_enum_maxval
      link override Signal_Limit/_minval: Value=KOUTP_AutoLTips_enum_minval
      link override Signal_Override/_ovrdflg: Value=KOUTP_AutoLTips_enum_ovrdflg
      link override Signal_Override/_ovrdval: Value=KOUTP_AutoLTips_enum_ovrdval
  VTPM_CWheelTips_enum_Inproc : FVT_lib/outp/OverrideAndLimit  SystemSampleTime=-1  VariantActivationTime=update diagram  Latency=0  AutoFrameSizeCalculation=off
      link override Signal_Limit/_maxval: Value=KOUTP_CWheelTips_enum_maxval
      link override Signal_Limit/_minval: Value=KOUTP_CWheelTips_enum_minval
      link override Signal_Override/_ovrdflg: Value=KOUTP_CWheelTips_enum_ovrdflg
      link override Signal_Override/_ovrdval: Value=KOUTP_CWheelTips_enum_ovrdval
  VTPM_ChkStorge_flg_Inproc : FVT_lib/outp/OverrideAndLimit  SystemSampleTime=-1  VariantActivationTime=update diagram  Latency=0  AutoFrameSizeCalculation=off
      link override Signal_Limit/_maxval: Value=KOUTP_ChkStorge_flg_maxval
      link override Signal_Limit/_minval: Value=KOUTP_ChkStorge_flg_minval
      link override Signal_Override/_ovrdflg: Value=KOUTP_ChkStorge_flg_ovrdflg
      link override Signal_Override/_ovrdval: Value=KOUTP_ChkStorge_flg_ovrdval
  VTPM_Chkfin_flg_Inproc : FVT_lib/outp/OverrideAndLimit  SystemSampleTime=-1  VariantActivationTime=update diagram  Latency=0  AutoFrameSizeCalculation=off
      link override Signal_Limit/_maxval: Value=KOUTP_Chkfin_flg_maxval
      link override Signal_Limit/_minval: Value=KOUTP_Chkfin_flg_minval
      link override Signal_Override/_ovrdflg: Value=KOUTP_Chkfin_flg_ovrdflg
      link override Signal_Override/_ovrdval: Value=KOUTP_Chkfin_flg_ovrdval
  VTPM_FAT_flg_Inproc : FVT_lib/outp/OverrideAndLimit  SystemSampleTime=-1  VariantActivationTime=update diagram  Latency=0  AutoFrameSizeCalculation=off
      link override Signal_Limit/_maxval: Value=KOUTP_FAT_flg_maxval
      link override Signal_Limit/_minval: Value=KOUTP_FAT_flg_minval
      link override Signal_Override/_ovrdflg: Value=KOUTP_FAT_flg_ovrdflg
      link override Signal_Override/_ovrdval: Value=KOUTP_FAT_flg_ovrdval
  VTPM_FlashIDvalid_enum_Inproc : FVT_lib/outp/OverrideAndLimit  SystemSampleTime=-1  VariantActivationTime=update diagram  Latency=0  AutoFrameSizeCalculation=off
      link override Signal_Limit/_maxval: Value=KOUTP_FlashIDvalid_enum_maxval
      link override Signal_Limit/_minval: Value=KOUTP_FlashIDvalid_enum_minval
      link override Signal_Override/_ovrdflg: Value=KOUTP_FlashIDvalid_enum_ovrdflg
      link override Signal_Override/_ovrdval: Value=KOUTP_FlashIDvalid_enum_ovrdval
  VTPM_FlashS1ID_raw_Inproc : FVT_lib/outp/OverrideAndLimit  SystemSampleTime=-1  VariantActivationTime=update diagram  Latency=0  AutoFrameSizeCalculation=off
      link override Signal_Limit/_maxval: Value=KOUTP_FlashS1ID_raw_maxval
      link override Signal_Limit/_minval: Value=KOUTP_FlashS1ID_raw_minval
      link override Signal_Override/_ovrdflg: Value=KOUTP_FlashS1ID_raw_ovrdflg
      link override Signal_Override/_ovrdval: Value=KOUTP_FlashS1ID_raw_ovrdval
  VTPM_FlashS2ID_raw_Inproc : FVT_lib/outp/OverrideAndLimit  SystemSampleTime=-1  VariantActivationTime=update diagram  Latency=0  AutoFrameSizeCalculation=off
      link override Signal_Limit/_maxval: Value=KOUTP_FlashS2ID_raw_maxval
      link override Signal_Limit/_minval: Value=KOUTP_FlashS2ID_raw_minval
      link override Signal_Override/_ovrdflg: Value=KOUTP_FlashS2ID_raw_ovrdflg
      link override Signal_Override/_ovrdval: Value=KOUTP_FlashS2ID_raw_ovrdval
  VTPM_FlashS3ID_raw_Inproc : FVT_lib/outp/OverrideAndLimit  SystemSampleTime=-1  VariantActivationTime=update diagram  Latency=0  AutoFrameSizeCalculation=off
      link override Signal_Limit/_maxval: Value=KOUTP_FlashS3ID_raw_maxval
      link override Signal_Limit/_minval: Value=KOUTP_FlashS3ID_raw_minval
      link override Signal_Override/_ovrdflg: Value=KOUTP_FlashS3ID_raw_ovrdflg
      link override Signal_Override/_ovrdval: Value=KOUTP_FlashS3ID_raw_ovrdval
  VTPM_FlashS4ID_raw_Inproc : FVT_lib/outp/OverrideAndLimit  SystemSampleTime=-1  VariantActivationTime=update diagram  Latency=0  AutoFrameSizeCalculation=off
      link override Signal_Limit/_maxval: Value=KOUTP_FlashS4ID_raw_maxval
      link override Signal_Limit/_minval: Value=KOUTP_FlashS4ID_raw_minval
      link override Signal_Override/_ovrdflg: Value=KOUTP_FlashS4ID_raw_ovrdflg
      link override Signal_Override/_ovrdval: Value=KOUTP_FlashS4ID_raw_ovrdval
  VTPM_Flashchkdatavalid_enum_Inproc : FVT_lib/outp/OverrideAndLimit  SystemSampleTime=-1  VariantActivationTime=update diagram  Latency=0  AutoFrameSizeCalculation=off
      link override Signal_Limit/_maxval: Value=KOUTP_Flashchkdatavalid_enum_maxval
      link override Signal_Limit/_minval: Value=KOUTP_Flashchkdatavalid_enum_minval
      link override Signal_Override/_ovrdflg: Value=KOUTP_Flashchkdatavalid_enum_ovrdflg
      link override Signal_Override/_ovrdval: Value=KOUTP_Flashchkdatavalid_enum_ovrdval
  VTPM_Flashdatavalid_enum_Inproc : FVT_lib/outp/OverrideAndLimit  SystemSampleTime=-1  VariantActivationTime=update diagram  Latency=0  AutoFrameSizeCalculation=off
      link override Signal_Limit/_maxval: Value=KOUTP_Flashdatavalid_enum_maxval
      link override Signal_Limit/_minval: Value=KOUTP_Flashdatavalid_enum_minval
      link override Signal_Override/_ovrdflg: Value=KOUTP_Flashdatavalid_enum_ovrdflg
      link override Signal_Override/_ovrdval: Value=KOUTP_Flashdatavalid_enum_ovrdval
  VTPM_ID1messageALTU_raw8_Inproc : FVT_lib/outp/OverrideAndLimit  SystemSampleTime=-1  VariantActivationTime=update diagram  Latency=0  AutoFrameSizeCalculation=off
      link override Signal_Limit/_maxval: Value=KOUTP_ID1messageALTU_raw8_maxval
      link override Signal_Limit/_minval: Value=KOUTP_ID1messageALTU_raw8_minval
      link override Signal_Override/_ovrdflg: Value=KOUTP_ID1messageALTU_raw8_ovrdflg
      link override Signal_Override/_ovrdval: Value=KOUTP_ID1messageALTU_raw8_ovrdval
  VTPM_ID2messageALTU_raw8_Inproc : FVT_lib/outp/OverrideAndLimit  SystemSampleTime=-1  VariantActivationTime=update diagram  Latency=0  AutoFrameSizeCalculation=off
      link override Signal_Limit/_maxval: Value=KOUTP_ID2messageALTU_raw8_maxval
      link override Signal_Limit/_minval: Value=KOUTP_ID2messageALTU_raw8_minval
      link override Signal_Override/_ovrdflg: Value=KOUTP_ID2messageALTU_raw8_ovrdflg
      link override Signal_Override/_ovrdval: Value=KOUTP_ID2messageALTU_raw8_ovrdval
  VTPM_ID3messageALTU_raw8_Inproc : FVT_lib/outp/OverrideAndLimit  SystemSampleTime=-1  VariantActivationTime=update diagram  Latency=0  AutoFrameSizeCalculation=off
      link override Signal_Limit/_maxval: Value=KOUTP_ID3messageALTU_raw8_maxval
      link override Signal_Limit/_minval: Value=KOUTP_ID3messageALTU_raw8_minval
      link override Signal_Override/_ovrdflg: Value=KOUTP_ID3messageALTU_raw8_ovrdflg
      link override Signal_Override/_ovrdval: Value=KOUTP_ID3messageALTU_raw8_ovrdval
  VTPM_ID4messageALTU_raw8_Inproc : FVT_lib/outp/OverrideAndLimit  SystemSampleTime=-1  VariantActivationTime=update diagram  Latency=0  AutoFrameSizeCalculation=off
      link override Signal_Limit/_maxval: Value=KOUTP_ID4messageALTU_raw8_maxval
      link override Signal_Limit/_minval: Value=KOUTP_ID4messageALTU_raw8_minval
      link override Signal_Override/_ovrdflg: Value=KOUTP_ID4messageALTU_raw8_ovrdflg
      link override Signal_Override/_ovrdval: Value=KOUTP_ID4messageALTU_raw8_ovrdval
  VTPM_IDin_raw32_Inproc : FVT_lib/outp/OverrideAndLimit  SystemSampleTime=-1  VariantActivationTime=update diagram  Latency=0  AutoFrameSizeCalculation=off
      link override Signal_Limit/_maxval: Value=KOUTP_IDin_raw32_maxval
      link override Signal_Limit/_minval: Value=KOUTP_IDin_raw32_minval
      link override Signal_Override/_ovrdflg: Value=KOUTP_IDin_raw32_ovrdflg
      link override Signal_Override/_ovrdval: Value=KOUTP_IDin_raw32_ovrdval
  VTPM_LFBatWarn_flg_Inproc : FVT_lib/outp/OverrideAndLimit  SystemSampleTime=-1  VariantActivationTime=update diagram  Latency=0  AutoFrameSizeCalculation=off
      link override Signal_Limit/_maxval: Value=KOUTP_LFBatWarn_flg_maxval
      link override Signal_Limit/_minval: Value=KOUTP_LFBatWarn_flg_minval
      link override Signal_Override/_ovrdflg: Value=KOUTP_LFBatWarn_flg_ovrdflg
      link override Signal_Override/_ovrdval: Value=KOUTP_LFBatWarn_flg_ovrdval
  VTPM_LFP20_raw8_Inproc : FVT_lib/outp/OverrideAndLimit  SystemSampleTime=-1  VariantActivationTime=update diagram  Latency=0  AutoFrameSizeCalculation=off
      link override Signal_Limit/_maxval: Value=KOUTP_LFP20_raw8_maxval
      link override Signal_Limit/_minval: Value=KOUTP_LFP20_raw8_minval
      link override Signal_Override/_ovrdflg: Value=KOUTP_LFP20_raw8_ovrdflg
      link override Signal_Override/_ovrdval: Value=KOUTP_LFP20_raw8_ovrdval
  VTPM_LFPindi_enum_Inproc : FVT_lib/outp/OverrideAndLimit  SystemSampleTime=-1  VariantActivationTime=update diagram  Latency=0  AutoFrameSizeCalculation=off
      link override Signal_Limit/_maxval: Value=KOUTP_LFPindi_enum_maxval
      link override Signal_Limit/_minval: Value=KOUTP_LFPindi_enum_minval
      link override Signal_Override/_ovrdflg: Value=KOUTP_LFPindi_enum_ovrdflg
      link override Signal_Override/_ovrdval: Value=KOUTP_LFPindi_enum_ovrdval
  VTPM_LFPressIndi_enum_Inproc : FVT_lib/outp/OverrideAndLimit  SystemSampleTime=-1  VariantActivationTime=update diagram  Latency=0  AutoFrameSizeCalculation=off
      link override Signal_Limit/_maxval: Value=KOUTP_LFPressIndi_enum_maxval
      link override Signal_Limit/_minval: Value=KOUTP_LFPressIndi_enum_minval
      link override Signal_Override/_ovrdflg: Value=KOUTP_LFPressIndi_enum_ovrdflg
      link override Signal_Override/_ovrdval: Value=KOUTP_LFPressIndi_enum_ovrdval
  VTPM_LFSensorFail_flg_Inproc : FVT_lib/outp/OverrideAndLimit  SystemSampleTime=-1  VariantActivationTime=update diagram  Latency=0  AutoFrameSizeCalculation=off
      link override Signal_Limit/_maxval: Value=KOUTP_LFSensorFail_flg_maxval
      link override Signal_Limit/_minval: Value=KOUTP_LFSensorFail_flg_minval
      link override Signal_Override/_ovrdflg: Value=KOUTP_LFSensorFail_flg_ovrdflg
      link override Signal_Override/_ovrdval: Value=KOUTP_LFSensorFail_flg_ovrdval
  VTPM_LFSensorMode_flg_Inproc : FVT_lib/outp/OverrideAndLimit  SystemSampleTime=-1  VariantActivationTime=update diagram  Latency=0  AutoFrameSizeCalculation=off
      link override Signal_Limit/_maxval: Value=KOUTP_LFSensorMode_flg_maxval
      link override Signal_Limit/_minval: Value=KOUTP_LFSensorMode_flg_minval
      link override Signal_Override/_ovrdflg: Value=KOUTP_LFSensorMode_flg_ovrdflg
      link override Signal_Override/_ovrdval: Value=KOUTP_LFSensorMode_flg_ovrdval
  VTPM_LFWheelDebug_flg_Inproc : FVT_lib/outp/OverrideAndLimit  SystemSampleTime=-1  VariantActivationTime=update diagram  Latency=0  AutoFrameSizeCalculation=off
      link override Signal_Limit/_maxval: Value=KOUTP_LFWheelDebug_flg_maxval
      link override Signal_Limit/_minval: Value=KOUTP_LFWheelDebug_flg_minval
      link override Signal_Override/_ovrdflg: Value=KOUTP_LFWheelDebug_flg_ovrdflg
      link override Signal_Override/_ovrdval: Value=KOUTP_LFWheelDebug_flg_ovrdval
  VTPM_LFWheelPSW_raw8_Inproc : FVT_lib/outp/OverrideAndLimit  SystemSampleTime=-1  VariantActivationTime=update diagram  Latency=0  AutoFrameSizeCalculation=off
      link override Signal_Limit/_maxval: Value=KOUTP_LFWheelPSW_raw8_maxval
      link override Signal_Limit/_minval: Value=KOUTP_LFWheelPSW_raw8_minval
      link override Signal_Override/_ovrdflg: Value=KOUTP_LFWheelPSW_raw8_ovrdflg
      link override Signal_Override/_ovrdval: Value=KOUTP_LFWheelPSW_raw8_ovrdval
  VTPM_LFWheelPress_raw8_Inproc : FVT_lib/outp/OverrideAndLimit  SystemSampleTime=-1  VariantActivationTime=update diagram  Latency=0  AutoFrameSizeCalculation=off
      link override Signal_Limit/_maxval: Value=KOUTP_LFWheelPress_raw8_maxval
      link override Signal_Limit/_minval: Value=KOUTP_LFWheelPress_raw8_minval
      link override Signal_Override/_ovrdflg: Value=KOUTP_LFWheelPress_raw8_ovrdflg
      link override Signal_Override/_ovrdval: Value=KOUTP_LFWheelPress_raw8_ovrdval
  VTPM_LFWheelTemp_C_Inproc : FVT_lib/outp/OverrideAndLimit  SystemSampleTime=-1  VariantActivationTime=update diagram  Latency=0  AutoFrameSizeCalculation=off
      link override Signal_Limit/_maxval: Value=KOUTP_LFWheelTemp_C_maxval
      link override Signal_Limit/_minval: Value=KOUTP_LFWheelTemp_C_minval
      link override Signal_Override/_ovrdflg: Value=KOUTP_LFWheelTemp_C_ovrdflg
      link override Signal_Override/_ovrdval: Value=KOUTP_LFWheelTemp_C_ovrdval
  VTPM_LFWheelTmpIndi_flg_Inproc : FVT_lib/outp/OverrideAndLimit  SystemSampleTime=-1  VariantActivationTime=update diagram  Latency=0  AutoFrameSizeCalculation=off
      link override Signal_Limit/_maxval: Value=KOUTP_LFWheelTmpIndi_flg_maxval
      link override Signal_Limit/_minval: Value=KOUTP_LFWheelTmpIndi_flg_minval
      link override Signal_Override/_ovrdflg: Value=KOUTP_LFWheelTmpIndi_flg_ovrdflg
      link override Signal_Override/_ovrdval: Value=KOUTP_LFWheelTmpIndi_flg_ovrdval
  VTPM_LProgress_enum_Inproc : FVT_lib/outp/OverrideAndLimit  SystemSampleTime=-1  VariantActivationTime=update diagram  Latency=0  AutoFrameSizeCalculation=off
      link override Signal_Limit/_maxval: Value=KOUTP_LProgress_enum_maxval
      link override Signal_Limit/_minval: Value=KOUTP_LProgress_enum_minval
      link override Signal_Override/_ovrdflg: Value=KOUTP_LProgress_enum_ovrdflg
      link override Signal_Override/_ovrdval: Value=KOUTP_LProgress_enum_ovrdval
  VTPM_LRBatWarn_flg_Inproc : FVT_lib/outp/OverrideAndLimit  SystemSampleTime=-1  VariantActivationTime=update diagram  Latency=0  AutoFrameSizeCalculation=off
      link override Signal_Limit/_maxval: Value=KOUTP_LRBatWarn_flg_maxval
      link override Signal_Limit/_minval: Value=KOUTP_LRBatWarn_flg_minval
      link override Signal_Override/_ovrdflg: Value=KOUTP_LRBatWarn_flg_ovrdflg
      link override Signal_Override/_ovrdval: Value=KOUTP_LRBatWarn_flg_ovrdval
  VTPM_LRP20_raw8_Inproc : FVT_lib/outp/OverrideAndLimit  SystemSampleTime=-1  VariantActivationTime=update diagram  Latency=0  AutoFrameSizeCalculation=off
      link override Signal_Limit/_maxval: Value=KOUTP_LRP20_raw8_maxval
      link override Signal_Limit/_minval: Value=KOUTP_LRP20_raw8_minval
      link override Signal_Override/_ovrdflg: Value=KOUTP_LRP20_raw8_ovrdflg
      link override Signal_Override/_ovrdval: Value=KOUTP_LRP20_raw8_ovrdval
  VTPM_LRPindi_enum_Inproc : FVT_lib/outp/OverrideAndLimit  SystemSampleTime=-1  VariantActivationTime=update diagram  Latency=0  AutoFrameSizeCalculation=off
      link override Signal_Limit/_maxval: Value=KOUTP_LRPindi_enum_maxval
      link override Signal_Limit/_minval: Value=KOUTP_LRPindi_enum_minval
      link override Signal_Override/_ovrdflg: Value=KOUTP_LRPindi_enum_ovrdflg
      link override Signal_Override/_ovrdval: Value=KOUTP_LRPindi_enum_ovrdval
  VTPM_LRPressIndi_enum_Inproc : FVT_lib/outp/OverrideAndLimit  SystemSampleTime=-1  VariantActivationTime=update diagram  Latency=0  AutoFrameSizeCalculation=off
      link override Signal_Limit/_maxval: Value=KOUTP_LRPressIndi_enum_maxval
      link override Signal_Limit/_minval: Value=KOUTP_LRPressIndi_enum_minval
      link override Signal_Override/_ovrdflg: Value=KOUTP_LRPressIndi_enum_ovrdflg
      link override Signal_Override/_ovrdval: Value=KOUTP_LRPressIndi_enum_ovrdval
  VTPM_LRSensorFail_flg_Inproc : FVT_lib/outp/OverrideAndLimit  SystemSampleTime=-1  VariantActivationTime=update diagram  Latency=0  AutoFrameSizeCalculation=off
      link override Signal_Limit/_maxval: Value=KOUTP_LRSensorFail_flg_maxval
      link override Signal_Limit/_minval: Value=KOUTP_LRSensorFail_flg_minval
      link override Signal_Override/_ovrdflg: Value=KOUTP_LRSensorFail_flg_ovrdflg
      link override Signal_Override/_ovrdval: Value=KOUTP_LRSensorFail_flg_ovrdval
  VTPM_LRSensorMode_flg_Inproc : FVT_lib/outp/OverrideAndLimit  SystemSampleTime=-1  VariantActivationTime=update diagram  Latency=0  AutoFrameSizeCalculation=off
      link override Signal_Limit/_maxval: Value=KOUTP_LRSensorMode_flg_maxval
      link override Signal_Limit/_minval: Value=KOUTP_LRSensorMode_flg_minval
      link override Signal_Override/_ovrdflg: Value=KOUTP_LRSensorMode_flg_ovrdflg
      link override Signal_Override/_ovrdval: Value=KOUTP_LRSensorMode_flg_ovrdval
  VTPM_LRWheelDebug_flg_Inproc : FVT_lib/outp/OverrideAndLimit  SystemSampleTime=-1  VariantActivationTime=update diagram  Latency=0  AutoFrameSizeCalculation=off
      link override Signal_Limit/_maxval: Value=KOUTP_LRWheelDebug_flg_maxval
      link override Signal_Limit/_minval: Value=KOUTP_LRWheelDebug_flg_minval
      link override Signal_Override/_ovrdflg: Value=KOUTP_LRWheelDebug_flg_ovrdflg
      link override Signal_Override/_ovrdval: Value=KOUTP_LRWheelDebug_flg_ovrdval
  VTPM_LRWheelPSW_raw8_Inproc : FVT_lib/outp/OverrideAndLimit  SystemSampleTime=-1  VariantActivationTime=update diagram  Latency=0  AutoFrameSizeCalculation=off
      link override Signal_Limit/_maxval: Value=KOUTP_LRWheelPSW_raw8_maxval
      link override Signal_Limit/_minval: Value=KOUTP_LRWheelPSW_raw8_minval
      link override Signal_Override/_ovrdflg: Value=KOUTP_LRWheelPSW_raw8_ovrdflg
      link override Signal_Override/_ovrdval: Value=KOUTP_LRWheelPSW_raw8_ovrdval
  VTPM_LRWheelPress_raw8_Inproc : FVT_lib/outp/OverrideAndLimit  SystemSampleTime=-1  VariantActivationTime=update diagram  Latency=0  AutoFrameSizeCalculation=off
      link override Signal_Limit/_maxval: Value=KOUTP_LRWheelPress_raw8_maxval
      link override Signal_Limit/_minval: Value=KOUTP_LRWheelPress_raw8_minval
      link override Signal_Override/_ovrdflg: Value=KOUTP_LRWheelPress_raw8_ovrdflg
      link override Signal_Override/_ovrdval: Value=KOUTP_LRWheelPress_raw8_ovrdval
  VTPM_LRWheelTemp_C_Inproc : FVT_lib/outp/OverrideAndLimit  SystemSampleTime=-1  VariantActivationTime=update diagram  Latency=0  AutoFrameSizeCalculation=off
      link override Signal_Limit/_maxval: Value=KOUTP_LRWheelTemp_C_maxval
      link override Signal_Limit/_minval: Value=KOUTP_LRWheelTemp_C_minval
      link override Signal_Override/_ovrdflg: Value=KOUTP_LRWheelTemp_C_ovrdflg
      link override Signal_Override/_ovrdval: Value=KOUTP_LRWheelTemp_C_ovrdval
  VTPM_LRWheelTmpIndi_flg_Inproc : FVT_lib/outp/OverrideAndLimit  SystemSampleTime=-1  VariantActivationTime=update diagram  Latency=0  AutoFrameSizeCalculation=off
      link override Signal_Limit/_maxval: Value=KOUTP_LRWheelTmpIndi_flg_maxval
      link override Signal_Limit/_minval: Value=KOUTP_LRWheelTmpIndi_flg_minval
      link override Signal_Override/_ovrdflg: Value=KOUTP_LRWheelTmpIndi_flg_ovrdflg
      link override Signal_Override/_ovrdval: Value=KOUTP_LRWheelTmpIndi_flg_ovrdval
  VTPM_ModelVersionChksum_raw_Inproc : FVT_lib/outp/OverrideAndLimit  SystemSampleTime=-1  VariantActivationTime=update diagram  Latency=0  AutoFrameSizeCalculation=off
      link override Signal_Limit/_maxval: Value=KOUTP_ModelVersionChksum_raw_maxval
      link override Signal_Limit/_minval: Value=KOUTP_ModelVersionChksum_raw_minval
      link override Signal_Override/_ovrdflg: Value=KOUTP_ModelVersionChksum_raw_ovrdflg
      link override Signal_Override/_ovrdval: Value=KOUTP_ModelVersionChksum_raw_ovrdval
  VTPM_ModelVersion_raw_Inproc : FVT_lib/outp/OverrideAndLimit  SystemSampleTime=-1  VariantActivationTime=update diagram  Latency=0  AutoFrameSizeCalculation=off
      link override Signal_Limit/_maxval: Value=KOUTP_ModelVersion_raw_maxval
      link override Signal_Limit/_minval: Value=KOUTP_ModelVersion_raw_minval
      link override Signal_Override/_ovrdflg: Value=KOUTP_ModelVersion_raw_ovrdflg
      link override Signal_Override/_ovrdval: Value=KOUTP_ModelVersion_raw_ovrdval
  VTPM_Prepresstempvalid_enum_Inproc : FVT_lib/outp/OverrideAndLimit  SystemSampleTime=-1  VariantActivationTime=update diagram  Latency=0  AutoFrameSizeCalculation=off
      link override Signal_Limit/_maxval: Value=KOUTP_Prepresstempvalid_enum_maxval
      link override Signal_Limit/_minval: Value=KOUTP_Prepresstempvalid_enum_minval
      link override Signal_Override/_ovrdflg: Value=KOUTP_Prepresstempvalid_enum_ovrdflg
      link override Signal_Override/_ovrdval: Value=KOUTP_Prepresstempvalid_enum_ovrdval
  VTPM_RFBatWarn_flg_Inproc : FVT_lib/outp/OverrideAndLimit  SystemSampleTime=-1  VariantActivationTime=update diagram  Latency=0  AutoFrameSizeCalculation=off
      link override Signal_Limit/_maxval: Value=KOUTP_RFBatWarn_flg_maxval
      link override Signal_Limit/_minval: Value=KOUTP_RFBatWarn_flg_minval
      link override Signal_Override/_ovrdflg: Value=KOUTP_RFBatWarn_flg_ovrdflg
      link override Signal_Override/_ovrdval: Value=KOUTP_RFBatWarn_flg_ovrdval
  VTPM_RFP20_raw8_Inproc : FVT_lib/outp/OverrideAndLimit  SystemSampleTime=-1  VariantActivationTime=update diagram  Latency=0  AutoFrameSizeCalculation=off
      link override Signal_Limit/_maxval: Value=KOUTP_RFP20_raw8_maxval
      link override Signal_Limit/_minval: Value=KOUTP_RFP20_raw8_minval
      link override Signal_Override/_ovrdflg: Value=KOUTP_RFP20_raw8_ovrdflg
      link override Signal_Override/_ovrdval: Value=KOUTP_RFP20_raw8_ovrdval
  VTPM_RFPind_enum_Inproc : FVT_lib/outp/OverrideAndLimit  SystemSampleTime=-1  VariantActivationTime=update diagram  Latency=0  AutoFrameSizeCalculation=off
      link override Signal_Limit/_maxval: Value=KOUTP_RFPind_enum_maxval
      link override Signal_Limit/_minval: Value=KOUTP_RFPind_enum_minval
      link override Signal_Override/_ovrdflg: Value=KOUTP_RFPind_enum_ovrdflg
      link override Signal_Override/_ovrdval: Value=KOUTP_RFPind_enum_ovrdval
  VTPM_RFPressIndi_enum_Inproc : FVT_lib/outp/OverrideAndLimit  SystemSampleTime=-1  VariantActivationTime=update diagram  Latency=0  AutoFrameSizeCalculation=off
      link override Signal_Limit/_maxval: Value=KOUTP_RFPressIndi_enum_maxval
      link override Signal_Limit/_minval: Value=KOUTP_RFPressIndi_enum_minval
      link override Signal_Override/_ovrdflg: Value=KOUTP_RFPressIndi_enum_ovrdflg
      link override Signal_Override/_ovrdval: Value=KOUTP_RFPressIndi_enum_ovrdval
  VTPM_RFSensorFail_flg_Inproc : FVT_lib/outp/OverrideAndLimit  SystemSampleTime=-1  VariantActivationTime=update diagram  Latency=0  AutoFrameSizeCalculation=off
      link override Signal_Limit/_maxval: Value=KOUTP_RFSensorFail_flg_maxval
      link override Signal_Limit/_minval: Value=KOUTP_RFSensorFail_flg_minval
      link override Signal_Override/_ovrdflg: Value=KOUTP_RFSensorFail_flg_ovrdflg
      link override Signal_Override/_ovrdval: Value=KOUTP_RFSensorFail_flg_ovrdval
  VTPM_RFSensorMode_flg_Inproc : FVT_lib/outp/OverrideAndLimit  SystemSampleTime=-1  VariantActivationTime=update diagram  Latency=0  AutoFrameSizeCalculation=off
      link override Signal_Limit/_maxval: Value=KOUTP_RFSensorMode_flg_maxval
      link override Signal_Limit/_minval: Value=KOUTP_RFSensorMode_flg_minval
      link override Signal_Override/_ovrdflg: Value=KOUTP_RFSensorMode_flg_ovrdflg
      link override Signal_Override/_ovrdval: Value=KOUTP_RFSensorMode_flg_ovrdval
  VTPM_RFWheelDebug_flg_Inproc : FVT_lib/outp/OverrideAndLimit  SystemSampleTime=-1  VariantActivationTime=update diagram  Latency=0  AutoFrameSizeCalculation=off
      link override Signal_Limit/_maxval: Value=KOUTP_RFWheelDebug_flg_maxval
      link override Signal_Limit/_minval: Value=KOUTP_RFWheelDebug_flg_minval
      link override Signal_Override/_ovrdflg: Value=KOUTP_RFWheelDebug_flg_ovrdflg
      link override Signal_Override/_ovrdval: Value=KOUTP_RFWheelDebug_flg_ovrdval
  VTPM_RFWheelPSW_raw8_Inproc : FVT_lib/outp/OverrideAndLimit  SystemSampleTime=-1  VariantActivationTime=update diagram  Latency=0  AutoFrameSizeCalculation=off
      link override Signal_Limit/_maxval: Value=KOUTP_RFWheelPSW_raw8_maxval
      link override Signal_Limit/_minval: Value=KOUTP_RFWheelPSW_raw8_minval
      link override Signal_Override/_ovrdflg: Value=KOUTP_RFWheelPSW_raw8_ovrdflg
      link override Signal_Override/_ovrdval: Value=KOUTP_RFWheelPSW_raw8_ovrdval
  VTPM_RFWheelPress_raw8_Inproc : FVT_lib/outp/OverrideAndLimit  SystemSampleTime=-1  VariantActivationTime=update diagram  Latency=0  AutoFrameSizeCalculation=off
      link override Signal_Limit/_maxval: Value=KOUTP_RFWheelPress_raw8_maxval
      link override Signal_Limit/_minval: Value=KOUTP_RFWheelPress_raw8_minval
      link override Signal_Override/_ovrdflg: Value=KOUTP_RFWheelPress_raw8_ovrdflg
      link override Signal_Override/_ovrdval: Value=KOUTP_RFWheelPress_raw8_ovrdval
  VTPM_RFWheelTemp_C_Inproc : FVT_lib/outp/OverrideAndLimit  SystemSampleTime=-1  VariantActivationTime=update diagram  Latency=0  AutoFrameSizeCalculation=off
      link override Signal_Limit/_maxval: Value=KOUTP_RFWheelTemp_C_maxval
      link override Signal_Limit/_minval: Value=KOUTP_RFWheelTemp_C_minval
      link override Signal_Override/_ovrdflg: Value=KOUTP_RFWheelTemp_C_ovrdflg
      link override Signal_Override/_ovrdval: Value=KOUTP_RFWheelTemp_C_ovrdval
  VTPM_RFWheelTmpIndi_flg_Inproc : FVT_lib/outp/OverrideAndLimit  SystemSampleTime=-1  VariantActivationTime=update diagram  Latency=0  AutoFrameSizeCalculation=off
      link override Signal_Limit/_maxval: Value=KOUTP_RFWheelTmpIndi_flg_maxval
      link override Signal_Limit/_minval: Value=KOUTP_RFWheelTmpIndi_flg_minval
      link override Signal_Override/_ovrdflg: Value=KOUTP_RFWheelTmpIndi_flg_ovrdflg
      link override Signal_Override/_ovrdval: Value=KOUTP_RFWheelTmpIndi_flg_ovrdval
  VTPM_RRBatWarn_flg_Inproc : FVT_lib/outp/OverrideAndLimit  SystemSampleTime=-1  VariantActivationTime=update diagram  Latency=0  AutoFrameSizeCalculation=off
      link override Signal_Limit/_maxval: Value=KOUTP_RRBatWarn_flg_maxval
      link override Signal_Limit/_minval: Value=KOUTP_RRBatWarn_flg_minval
      link override Signal_Override/_ovrdflg: Value=KOUTP_RRBatWarn_flg_ovrdflg
      link override Signal_Override/_ovrdval: Value=KOUTP_RRBatWarn_flg_ovrdval
  VTPM_RRP20_raw8_Inproc : FVT_lib/outp/OverrideAndLimit  SystemSampleTime=-1  VariantActivationTime=update diagram  Latency=0  AutoFrameSizeCalculation=off
      link override Signal_Limit/_maxval: Value=KOUTP_RRP20_raw8_maxval
      link override Signal_Limit/_minval: Value=KOUTP_RRP20_raw8_minval
      link override Signal_Override/_ovrdflg: Value=KOUTP_RRP20_raw8_ovrdflg
      link override Signal_Override/_ovrdval: Value=KOUTP_RRP20_raw8_ovrdval
  VTPM_RRPindi_enum_Inproc : FVT_lib/outp/OverrideAndLimit  SystemSampleTime=-1  VariantActivationTime=update diagram  Latency=0  AutoFrameSizeCalculation=off
      link override Signal_Limit/_maxval: Value=KOUTP_RRPindi_enum_maxval
      link override Signal_Limit/_minval: Value=KOUTP_RRPindi_enum_minval
      link override Signal_Override/_ovrdflg: Value=KOUTP_RRPindi_enum_ovrdflg
      link override Signal_Override/_ovrdval: Value=KOUTP_RRPindi_enum_ovrdval
  VTPM_RRPressIndi_enum_Inproc : FVT_lib/outp/OverrideAndLimit  SystemSampleTime=-1  VariantActivationTime=update diagram  Latency=0  AutoFrameSizeCalculation=off
      link override Signal_Limit/_maxval: Value=KOUTP_RRPressIndi_enum_maxval
      link override Signal_Limit/_minval: Value=KOUTP_RRPressIndi_enum_minval
      link override Signal_Override/_ovrdflg: Value=KOUTP_RRPressIndi_enum_ovrdflg
      link override Signal_Override/_ovrdval: Value=KOUTP_RRPressIndi_enum_ovrdval
  VTPM_RRSensorFail_flg_Inproc : FVT_lib/outp/OverrideAndLimit  SystemSampleTime=-1  VariantActivationTime=update diagram  Latency=0  AutoFrameSizeCalculation=off
      link override Signal_Limit/_maxval: Value=KOUTP_RRSensorFail_flg_maxval
      link override Signal_Limit/_minval: Value=KOUTP_RRSensorFail_flg_minval
      link override Signal_Override/_ovrdflg: Value=KOUTP_RRSensorFail_flg_ovrdflg
      link override Signal_Override/_ovrdval: Value=KOUTP_RRSensorFail_flg_ovrdval
  VTPM_RRSensorMode_flg_Inproc : FVT_lib/outp/OverrideAndLimit  SystemSampleTime=-1  VariantActivationTime=update diagram  Latency=0  AutoFrameSizeCalculation=off
      link override Signal_Limit/_maxval: Value=KOUTP_RRSensorMode_flg_maxval
      link override Signal_Limit/_minval: Value=KOUTP_RRSensorMode_flg_minval
      link override Signal_Override/_ovrdflg: Value=KOUTP_RRSensorMode_flg_ovrdflg
      link override Signal_Override/_ovrdval: Value=KOUTP_RRSensorMode_flg_ovrdval
  VTPM_RRWheelDebug_flg_Inproc : FVT_lib/outp/OverrideAndLimit  SystemSampleTime=-1  VariantActivationTime=update diagram  Latency=0  AutoFrameSizeCalculation=off
      link override Signal_Limit/_maxval: Value=KOUTP_RRWheelDebug_flg_maxval
      link override Signal_Limit/_minval: Value=KOUTP_RRWheelDebug_flg_minval
      link override Signal_Override/_ovrdflg: Value=KOUTP_RRWheelDebug_flg_ovrdflg
      link override Signal_Override/_ovrdval: Value=KOUTP_RRWheelDebug_flg_ovrdval
  VTPM_RRWheelPSW_raw8_Inproc : FVT_lib/outp/OverrideAndLimit  SystemSampleTime=-1  VariantActivationTime=update diagram  Latency=0  AutoFrameSizeCalculation=off
      link override Signal_Limit/_maxval: Value=KOUTP_RRWheelPSW_raw8_maxval
      link override Signal_Limit/_minval: Value=KOUTP_RRWheelPSW_raw8_minval
      link override Signal_Override/_ovrdflg: Value=KOUTP_RRWheelPSW_raw8_ovrdflg
      link override Signal_Override/_ovrdval: Value=KOUTP_RRWheelPSW_raw8_ovrdval
  VTPM_RRWheelPress_raw8_Inproc : FVT_lib/outp/OverrideAndLimit  SystemSampleTime=-1  VariantActivationTime=update diagram  Latency=0  AutoFrameSizeCalculation=off
      link override Signal_Limit/_maxval: Value=KOUTP_RRWheelPress_raw8_maxval
      link override Signal_Limit/_minval: Value=KOUTP_RRWheelPress_raw8_minval
      link override Signal_Override/_ovrdflg: Value=KOUTP_RRWheelPress_raw8_ovrdflg
      link override Signal_Override/_ovrdval: Value=KOUTP_RRWheelPress_raw8_ovrdval
  VTPM_RRWheelTemp_C_Inproc : FVT_lib/outp/OverrideAndLimit  SystemSampleTime=-1  VariantActivationTime=update diagram  Latency=0  AutoFrameSizeCalculation=off
      link override Signal_Limit/_maxval: Value=KOUTP_RRWheelTemp_C_maxval
      link override Signal_Limit/_minval: Value=KOUTP_RRWheelTemp_C_minval
      link override Signal_Override/_ovrdflg: Value=KOUTP_RRWheelTemp_C_ovrdflg
      link override Signal_Override/_ovrdval: Value=KOUTP_RRWheelTemp_C_ovrdval
  VTPM_RRWheelTmpIndi_flg_Inproc : FVT_lib/outp/OverrideAndLimit  SystemSampleTime=-1  VariantActivationTime=update diagram  Latency=0  AutoFrameSizeCalculation=off
      link override Signal_Limit/_maxval: Value=KOUTP_RRWheelTmpIndi_flg_maxval
      link override Signal_Limit/_minval: Value=KOUTP_RRWheelTmpIndi_flg_minval
      link override Signal_Override/_ovrdflg: Value=KOUTP_RRWheelTmpIndi_flg_ovrdflg
      link override Signal_Override/_ovrdval: Value=KOUTP_RRWheelTmpIndi_flg_ovrdval
  VTPM_S1ID_raw32_Inproc : FVT_lib/outp/OverrideAndLimit  SystemSampleTime=-1  VariantActivationTime=update diagram  Latency=0  AutoFrameSizeCalculation=off
      link override Signal_Limit/_maxval: Value=KOUTP_S1ID_raw32_maxval
      link override Signal_Limit/_minval: Value=KOUTP_S1ID_raw32_minval
      link override Signal_Override/_ovrdflg: Value=KOUTP_S1ID_raw32_ovrdflg
      link override Signal_Override/_ovrdval: Value=KOUTP_S1ID_raw32_ovrdval
  VTPM_S1L_enum_Inproc : FVT_lib/outp/OverrideAndLimit  SystemSampleTime=-1  VariantActivationTime=update diagram  Latency=0  AutoFrameSizeCalculation=off
      link override Signal_Limit/_maxval: Value=KOUTP_S1L_enum_maxval
      link override Signal_Limit/_minval: Value=KOUTP_S1L_enum_minval
      link override Signal_Override/_ovrdflg: Value=KOUTP_S1L_enum_ovrdflg
      link override Signal_Override/_ovrdval: Value=KOUTP_S1L_enum_ovrdval
  VTPM_S1WheelDebugALTU_pct_Inproc : FVT_lib/outp/OverrideAndLimit  SystemSampleTime=-1  VariantActivationTime=update diagram  Latency=0  AutoFrameSizeCalculation=off
      link override Signal_Limit/_maxval: Value=KOUTP_S1WheelDebugALTU_pct_maxval
      link override Signal_Limit/_minval: Value=KOUTP_S1WheelDebugALTU_pct_minval
      link override Signal_Override/_ovrdflg: Value=KOUTP_S1WheelDebugALTU_pct_ovrdflg
      link override Signal_Override/_ovrdval: Value=KOUTP_S1WheelDebugALTU_pct_ovrdval
  VTPM_S2ID_raw32_Inproc : FVT_lib/outp/OverrideAndLimit  SystemSampleTime=-1  VariantActivationTime=update diagram  Latency=0  AutoFrameSizeCalculation=off
      link override Signal_Limit/_maxval: Value=KOUTP_S2ID_raw32_maxval
      link override Signal_Limit/_minval: Value=KOUTP_S2ID_raw32_minval
      link override Signal_Override/_ovrdflg: Value=KOUTP_S2ID_raw32_ovrdflg
      link override Signal_Override/_ovrdval: Value=KOUTP_S2ID_raw32_ovrdval
  VTPM_S2L_enum_Inproc : FVT_lib/outp/OverrideAndLimit  SystemSampleTime=-1  VariantActivationTime=update diagram  Latency=0  AutoFrameSizeCalculation=off
      link override Signal_Limit/_maxval: Value=KOUTP_S2L_enum_maxval
      link override Signal_Limit/_minval: Value=KOUTP_S2L_enum_minval
      link override Signal_Override/_ovrdflg: Value=KOUTP_S2L_enum_ovrdflg
      link override Signal_Override/_ovrdval: Value=KOUTP_S2L_enum_ovrdval
  VTPM_S2WheelDebugALTU_pct_Inproc : FVT_lib/outp/OverrideAndLimit  SystemSampleTime=-1  VariantActivationTime=update diagram  Latency=0  AutoFrameSizeCalculation=off
      link override Signal_Limit/_maxval: Value=KOUTP_S2WheelDebugALTU_pct_maxval
      link override Signal_Limit/_minval: Value=KOUTP_S2WheelDebugALTU_pct_minval
      link override Signal_Override/_ovrdflg: Value=KOUTP_S2WheelDebugALTU_pct_ovrdflg
      link override Signal_Override/_ovrdval: Value=KOUTP_S2WheelDebugALTU_pct_ovrdval
  VTPM_S3ID_raw32_Inproc : FVT_lib/outp/OverrideAndLimit  SystemSampleTime=-1  VariantActivationTime=update diagram  Latency=0  AutoFrameSizeCalculation=off
      link override Signal_Limit/_maxval: Value=KOUTP_S3ID_raw32_maxval
      link override Signal_Limit/_minval: Value=KOUTP_S3ID_raw32_minval
      link override Signal_Override/_ovrdflg: Value=KOUTP_S3ID_raw32_ovrdflg
      link override Signal_Override/_ovrdval: Value=KOUTP_S3ID_raw32_ovrdval
  VTPM_S3L_enum_Inproc : FVT_lib/outp/OverrideAndLimit  SystemSampleTime=-1  VariantActivationTime=update diagram  Latency=0  AutoFrameSizeCalculation=off
      link override Signal_Limit/_maxval: Value=KOUTP_S3L_enum_maxval
      link override Signal_Limit/_minval: Value=KOUTP_S3L_enum_minval
      link override Signal_Override/_ovrdflg: Value=KOUTP_S3L_enum_ovrdflg
      link override Signal_Override/_ovrdval: Value=KOUTP_S3L_enum_ovrdval
  VTPM_S3WheelDebugALTU_pct_Inproc : FVT_lib/outp/OverrideAndLimit  SystemSampleTime=-1  VariantActivationTime=update diagram  Latency=0  AutoFrameSizeCalculation=off
      link override Signal_Limit/_maxval: Value=KOUTP_S3WheelDebugALTU_pct_maxval
      link override Signal_Limit/_minval: Value=KOUTP_S3WheelDebugALTU_pct_minval
      link override Signal_Override/_ovrdflg: Value=KOUTP_S3WheelDebugALTU_pct_ovrdflg
      link override Signal_Override/_ovrdval: Value=KOUTP_S3WheelDebugALTU_pct_ovrdval
  VTPM_S4ID_raw32_Inproc : FVT_lib/outp/OverrideAndLimit  SystemSampleTime=-1  VariantActivationTime=update diagram  Latency=0  AutoFrameSizeCalculation=off
      link override Signal_Limit/_maxval: Value=KOUTP_S4ID_raw32_maxval
      link override Signal_Limit/_minval: Value=KOUTP_S4ID_raw32_minval
      link override Signal_Override/_ovrdflg: Value=KOUTP_S4ID_raw32_ovrdflg
      link override Signal_Override/_ovrdval: Value=KOUTP_S4ID_raw32_ovrdval
  VTPM_S4L_enum_Inproc : FVT_lib/outp/OverrideAndLimit  SystemSampleTime=-1  VariantActivationTime=update diagram  Latency=0  AutoFrameSizeCalculation=off
      link override Signal_Limit/_maxval: Value=KOUTP_S4L_enum_maxval
      link override Signal_Limit/_minval: Value=KOUTP_S4L_enum_minval
      link override Signal_Override/_ovrdflg: Value=KOUTP_S4L_enum_ovrdflg
      link override Signal_Override/_ovrdval: Value=KOUTP_S4L_enum_ovrdval
  VTPM_S4WheelDebugALTU_pct_Inproc : FVT_lib/outp/OverrideAndLimit  SystemSampleTime=-1  VariantActivationTime=update diagram  Latency=0  AutoFrameSizeCalculation=off
      link override Signal_Limit/_maxval: Value=KOUTP_S4WheelDebugALTU_pct_maxval
      link override Signal_Limit/_minval: Value=KOUTP_S4WheelDebugALTU_pct_minval
      link override Signal_Override/_ovrdflg: Value=KOUTP_S4WheelDebugALTU_pct_ovrdflg
      link override Signal_Override/_ovrdval: Value=KOUTP_S4WheelDebugALTU_pct_ovrdval
  VTPM_SetIDLoc_flg_Inproc : FVT_lib/outp/OverrideAndLimit  SystemSampleTime=-1  VariantActivationTime=update diagram  Latency=0  AutoFrameSizeCalculation=off
      link override Signal_Limit/_maxval: Value=KOUTP_SetIDLoc_flg_maxval
      link override Signal_Limit/_minval: Value=KOUTP_SetIDLoc_flg_minval
      link override Signal_Override/_ovrdflg: Value=KOUTP_SetIDLoc_flg_ovrdflg
      link override Signal_Override/_ovrdval: Value=KOUTP_SetIDLoc_flg_ovrdval
  VTPM_TPMSCaliButtAllow_flg_Inproc : FVT_lib/outp/OverrideAndLimit  SystemSampleTime=-1  VariantActivationTime=update diagram  Latency=0  AutoFrameSizeCalculation=off
      link override Signal_Limit/_maxval: Value=KOUTP_TPMSCaliButtAllow_flg_maxval
      link override Signal_Limit/_minval: Value=KOUTP_TPMSCaliButtAllow_flg_minval
      link override Signal_Override/_ovrdflg: Value=KOUTP_TPMSCaliButtAllow_flg_ovrdflg
      link override Signal_Override/_ovrdval: Value=KOUTP_TPMSCaliButtAllow_flg_ovrdval
  VTPM_TPMSResButtAllow_flg_Inproc : FVT_lib/outp/OverrideAndLimit  SystemSampleTime=-1  VariantActivationTime=update diagram  Latency=0  AutoFrameSizeCalculation=off
      link override Signal_Limit/_maxval: Value=KOUTP_TPMSResButtAllow_flg_maxval
      link override Signal_Limit/_minval: Value=KOUTP_TPMSResButtAllow_flg_minval
      link override Signal_Override/_ovrdflg: Value=KOUTP_TPMSResButtAllow_flg_ovrdflg
      link override Signal_Override/_ovrdval: Value=KOUTP_TPMSResButtAllow_flg_ovrdval
  VTPM_TPMSResButt_flg_Inproc : FVT_lib/outp/OverrideAndLimit  SystemSampleTime=-1  VariantActivationTime=update diagram  Latency=0  AutoFrameSizeCalculation=off
      link override Signal_Limit/_maxval: Value=KOUTP_TPMSResButt_flg_maxval
      link override Signal_Limit/_minval: Value=KOUTP_TPMSResButt_flg_minval
      link override Signal_Override/_ovrdflg: Value=KOUTP_TPMSResButt_flg_ovrdflg
      link override Signal_Override/_ovrdval: Value=KOUTP_TPMSResButt_flg_ovrdval
  VTPM_TPMSSensorIDRegStart_flg_Inproc : FVT_lib/outp/OverrideAndLimit  SystemSampleTime=-1  VariantActivationTime=update diagram  Latency=0  AutoFrameSizeCalculation=off
      link override Signal_Limit/_maxval: Value=KOUTP_TPMSSensorIDRegStart_flg_maxval
      link override Signal_Limit/_minval: Value=KOUTP_TPMSSensorIDRegStart_flg_minval
      link override Signal_Override/_ovrdflg: Value=KOUTP_TPMSSensorIDRegStart_flg_ovrdflg
      link override Signal_Override/_ovrdval: Value=KOUTP_TPMSSensorIDRegStart_flg_ovrdval
  VTPM_TPMSStorge_flg_Inproc : FVT_lib/outp/OverrideAndLimit  SystemSampleTime=-1  VariantActivationTime=update diagram  Latency=0  AutoFrameSizeCalculation=off
      link override Signal_Limit/_maxval: Value=KOUTP_TPMSStorge_flg_maxval
      link override Signal_Limit/_minval: Value=KOUTP_TPMSStorge_flg_minval
      link override Signal_Override/_ovrdflg: Value=KOUTP_TPMSStorge_flg_ovrdflg
      link override Signal_Override/_ovrdval: Value=KOUTP_TPMSStorge_flg_ovrdval
  VTPM_TPMSTLCmd_flg_Inproc : FVT_lib/outp/OverrideAndLimit  SystemSampleTime=-1  VariantActivationTime=update diagram  Latency=0  AutoFrameSizeCalculation=off
      link override Signal_Limit/_maxval: Value=KOUTP_TPMSTLCmd_flg_maxval
      link override Signal_Limit/_minval: Value=KOUTP_TPMSTLCmd_flg_minval
      link override Signal_Override/_ovrdflg: Value=KOUTP_TPMSTLCmd_flg_ovrdflg
      link override Signal_Override/_ovrdval: Value=KOUTP_TPMSTLCmd_flg_ovrdval
  VTPM_TPMSWarnIndi_enum_Inproc : FVT_lib/outp/OverrideAndLimit  SystemSampleTime=-1  VariantActivationTime=update diagram  Latency=0  AutoFrameSizeCalculation=off
      link override Signal_Limit/_maxval: Value=KOUTP_TPMSWarnIndi_enum_maxval
      link override Signal_Limit/_minval: Value=KOUTP_TPMSWarnIndi_enum_minval
      link override Signal_Override/_ovrdflg: Value=KOUTP_TPMSWarnIndi_enum_ovrdflg
      link override Signal_Override/_ovrdval: Value=KOUTP_TPMSWarnIndi_enum_ovrdval
  VTPM_WriteChkLFID_raw_Inproc : FVT_lib/outp/OverrideAndLimit  SystemSampleTime=-1  VariantActivationTime=update diagram  Latency=0  AutoFrameSizeCalculation=off
      link override Signal_Limit/_maxval: Value=KOUTP_WriteChkLFID_raw_maxval
      link override Signal_Limit/_minval: Value=KOUTP_WriteChkLFID_raw_minval
      link override Signal_Override/_ovrdflg: Value=KOUTP_WriteChkLFID_raw_ovrdflg
      link override Signal_Override/_ovrdval: Value=KOUTP_WriteChkLFID_raw_ovrdval
  VTPM_WriteChkLRID_raw_Inproc : FVT_lib/outp/OverrideAndLimit  SystemSampleTime=-1  VariantActivationTime=update diagram  Latency=0  AutoFrameSizeCalculation=off
      link override Signal_Limit/_maxval: Value=KOUTP_WriteChkLRID_raw_maxval
      link override Signal_Limit/_minval: Value=KOUTP_WriteChkLRID_raw_minval
      link override Signal_Override/_ovrdflg: Value=KOUTP_WriteChkLRID_raw_ovrdflg
      link override Signal_Override/_ovrdval: Value=KOUTP_WriteChkLRID_raw_ovrdval
  VTPM_WriteChkRFID_raw_Inproc : FVT_lib/outp/OverrideAndLimit  SystemSampleTime=-1  VariantActivationTime=update diagram  Latency=0  AutoFrameSizeCalculation=off
      link override Signal_Limit/_maxval: Value=KOUTP_WriteChkRFID_raw_maxval
      link override Signal_Limit/_minval: Value=KOUTP_WriteChkRFID_raw_minval
      link override Signal_Override/_ovrdflg: Value=KOUTP_WriteChkRFID_raw_ovrdflg
      link override Signal_Override/_ovrdval: Value=KOUTP_WriteChkRFID_raw_ovrdval
  VTPM_WriteChkRRID_raw_Inproc : FVT_lib/outp/OverrideAndLimit  SystemSampleTime=-1  VariantActivationTime=update diagram  Latency=0  AutoFrameSizeCalculation=off
      link override Signal_Limit/_maxval: Value=KOUTP_WriteChkRRID_raw_maxval
      link override Signal_Limit/_minval: Value=KOUTP_WriteChkRRID_raw_minval
      link override Signal_Override/_ovrdflg: Value=KOUTP_WriteChkRRID_raw_ovrdflg
      link override Signal_Override/_ovrdval: Value=KOUTP_WriteChkRRID_raw_ovrdval
  VTPM_WriteChkfinLFID_raw_Inproc : FVT_lib/outp/OverrideAndLimit  SystemSampleTime=-1  VariantActivationTime=update diagram  Latency=0  AutoFrameSizeCalculation=off
      link override Signal_Limit/_maxval: Value=KOUTP_WriteChkfinLFID_raw_maxval
      link override Signal_Limit/_minval: Value=KOUTP_WriteChkfinLFID_raw_minval
      link override Signal_Override/_ovrdflg: Value=KOUTP_WriteChkfinLFID_raw_ovrdflg
      link override Signal_Override/_ovrdval: Value=KOUTP_WriteChkfinLFID_raw_ovrdval
  VTPM_WriteChkfinLRID_raw_Inproc : FVT_lib/outp/OverrideAndLimit  SystemSampleTime=-1  VariantActivationTime=update diagram  Latency=0  AutoFrameSizeCalculation=off
      link override Signal_Limit/_maxval: Value=KOUTP_WriteChkfinLRID_raw_maxval
      link override Signal_Limit/_minval: Value=KOUTP_WriteChkfinLRID_raw_minval
      link override Signal_Override/_ovrdflg: Value=KOUTP_WriteChkfinLRID_raw_ovrdflg
      link override Signal_Override/_ovrdval: Value=KOUTP_WriteChkfinLRID_raw_ovrdval
  VTPM_WriteChkfinRFID_raw_Inproc : FVT_lib/outp/OverrideAndLimit  SystemSampleTime=-1  VariantActivationTime=update diagram  Latency=0  AutoFrameSizeCalculation=off
      link override Signal_Limit/_maxval: Value=KOUTP_WriteChkfinRFID_raw_maxval
      link override Signal_Limit/_minval: Value=KOUTP_WriteChkfinRFID_raw_minval
      link override Signal_Override/_ovrdflg: Value=KOUTP_WriteChkfinRFID_raw_ovrdflg
      link override Signal_Override/_ovrdval: Value=KOUTP_WriteChkfinRFID_raw_ovrdval
  VTPM_WriteChkfinRRID_raw_Inproc : FVT_lib/outp/OverrideAndLimit  SystemSampleTime=-1  VariantActivationTime=update diagram  Latency=0  AutoFrameSizeCalculation=off
      link override Signal_Limit/_maxval: Value=KOUTP_WriteChkfinRRID_raw_maxval
      link override Signal_Limit/_minval: Value=KOUTP_WriteChkfinRRID_raw_minval
      link override Signal_Override/_ovrdflg: Value=KOUTP_WriteChkfinRRID_raw_ovrdflg
      link override Signal_Override/_ovrdval: Value=KOUTP_WriteChkfinRRID_raw_ovrdval
  VTPM_WritingCnt_enum_Inproc : FVT_lib/outp/OverrideAndLimit  SystemSampleTime=-1  VariantActivationTime=update diagram  Latency=0  AutoFrameSizeCalculation=off
      link override Signal_Limit/_maxval: Value=KOUTP_WritingCnt_enum_maxval
      link override Signal_Limit/_minval: Value=KOUTP_WritingCnt_enum_minval
      link override Signal_Override/_ovrdflg: Value=KOUTP_WritingCnt_enum_ovrdflg
      link override Signal_Override/_ovrdval: Value=KOUTP_WritingCnt_enum_ovrdval
  VTPM_unlearnSfailvalid_enum_Inproc : FVT_lib/outp/OverrideAndLimit  SystemSampleTime=-1  VariantActivationTime=update diagram  Latency=0  AutoFrameSizeCalculation=off
      link override Signal_Limit/_maxval: Value=KOUTP_unlearnSfailvalid_enum_maxval
      link override Signal_Limit/_minval: Value=KOUTP_unlearnSfailvalid_enum_minval
      link override Signal_Override/_ovrdflg: Value=KOUTP_unlearnSfailvalid_enum_ovrdflg
      link override Signal_Override/_ovrdval: Value=KOUTP_unlearnSfailvalid_enum_ovrdval
  VTPM_unlearnSfali_flg_Inproc : FVT_lib/outp/OverrideAndLimit  SystemSampleTime=-1  VariantActivationTime=update diagram  Latency=0  AutoFrameSizeCalculation=off
      link override Signal_Limit/_maxval: Value=KOUTP_unlearnSfali_flg_maxval
      link override Signal_Limit/_minval: Value=KOUTP_unlearnSfali_flg_minval
      link override Signal_Override/_ovrdflg: Value=KOUTP_unlearnSfali_flg_ovrdflg
      link override Signal_Override/_ovrdval: Value=KOUTP_unlearnSfali_flg_ovrdval
  VTQD_ActParkRequest_flg_Inproc : FVT_lib/outp/OverrideAndLimit  SystemSampleTime=-1  VariantActivationTime=update diagram  Latency=0  AutoFrameSizeCalculation=off
      link override Signal_Limit/_maxval: Value=KOUTP_ActParkRequest_flg_maxval
      link override Signal_Limit/_minval: Value=KOUTP_ActParkRequest_flg_minval
      link override Signal_Override/_ovrdflg: Value=KOUTP_ActParkRequest_flg_ovrdflg
      link override Signal_Override/_ovrdval: Value=KOUTP_ActParkRequest_flg_ovrdval
  VTQD_CreepON_flg_Inproc : FVT_lib/outp/OverrideAndLimit  SystemSampleTime=-1  VariantActivationTime=update diagram  Latency=0  AutoFrameSizeCalculation=off
      link override Signal_Limit/_maxval: Value=KOUTP_CreepON_flg_maxval
      link override Signal_Limit/_minval: Value=KOUTP_CreepON_flg_minval
      link override Signal_Override/_ovrdflg: Value=KOUTP_CreepON_flg_ovrdflg
      link override Signal_Override/_ovrdval: Value=KOUTP_CreepON_flg_ovrdval
  VTQD_DriveProtEn_flg_Inproc : FVT_lib/outp/OverrideAndLimit  SystemSampleTime=-1  VariantActivationTime=update diagram  Latency=0  AutoFrameSizeCalculation=off
      link override Signal_Limit/_maxval: Value=KOUTP_DriveProtEn_flg_maxval
      link override Signal_Limit/_minval: Value=KOUTP_DriveProtEn_flg_minval
      link override Signal_Override/_ovrdflg: Value=KOUTP_DriveProtEn_flg_ovrdflg
      link override Signal_Override/_ovrdval: Value=KOUTP_DriveProtEn_flg_ovrdval
  VTQD_DriverWhlTqDemFr_Nm_Inproc : FVT_lib/outp/OverrideAndLimit  SystemSampleTime=-1  VariantActivationTime=update diagram  Latency=0  AutoFrameSizeCalculation=off
      link override Signal_Limit/_maxval: Value=KOUTP_DriverWhlTqDemFr_Nm_maxval
      link override Signal_Limit/_minval: Value=KOUTP_DriverWhlTqDemFr_Nm_minval
      link override Signal_Override/_ovrdflg: Value=KOUTP_DriverWhlTqDemFr_Nm_ovrdflg
      link override Signal_Override/_ovrdval: Value=KOUTP_DriverWhlTqDemFr_Nm_ovrdval
  VTQD_DriverWhlTqDemRr_Nm_Inproc : FVT_lib/outp/OverrideAndLimit  SystemSampleTime=-1  VariantActivationTime=update diagram  Latency=0  AutoFrameSizeCalculation=off
      link override Signal_Limit/_maxval: Value=KOUTP_DriverWhlTqDemRr_Nm_maxval
      link override Signal_Limit/_minval: Value=KOUTP_DriverWhlTqDemRr_Nm_minval
      link override Signal_Override/_ovrdflg: Value=KOUTP_DriverWhlTqDemRr_Nm_ovrdflg
      link override Signal_Override/_ovrdval: Value=KOUTP_DriverWhlTqDemRr_Nm_ovrdval
  VTQD_EVDriveMode_enum_Inproc : FVT_lib/outp/OverrideAndLimit  SystemSampleTime=-1  VariantActivationTime=update diagram  Latency=0  AutoFrameSizeCalculation=off
      link override Signal_Limit/_maxval: Value=KOUTP_EVDriveMode_enum_maxval
      link override Signal_Limit/_minval: Value=KOUTP_EVDriveMode_enum_minval
      link override Signal_Override/_ovrdflg: Value=KOUTP_EVDriveMode_enum_ovrdflg
      link override Signal_Override/_ovrdval: Value=KOUTP_EVDriveMode_enum_ovrdval
  VTQD_EquivAccPedalSWSta_flg_Inproc : FVT_lib/outp/OverrideAndLimit  SystemSampleTime=-1  VariantActivationTime=update diagram  Latency=0  AutoFrameSizeCalculation=off
      link override Signal_Limit/_maxval: Value=KOUTP_EquivAccPedalSWSta_flg_maxval
      link override Signal_Limit/_minval: Value=KOUTP_EquivAccPedalSWSta_flg_minval
      link override Signal_Override/_ovrdflg: Value=KOUTP_EquivAccPedalSWSta_flg_ovrdflg
      link override Signal_Override/_ovrdval: Value=KOUTP_EquivAccPedalSWSta_flg_ovrdval
  VTQD_FDCVCURegenMode_enum_Inproc : FVT_lib/outp/OverrideAndLimit  SystemSampleTime=-1  VariantActivationTime=update diagram  Latency=0  AutoFrameSizeCalculation=off
      link override Signal_Limit/_maxval: Value=KOUTP_FDCVCURegenMode_enum_maxval
      link override Signal_Limit/_minval: Value=KOUTP_FDCVCURegenMode_enum_minval
      link override Signal_Override/_ovrdflg: Value=KOUTP_FDCVCURegenMode_enum_ovrdflg
      link override Signal_Override/_ovrdval: Value=KOUTP_FDCVCURegenMode_enum_ovrdval
  VTQD_FrActvDmpDisabReq_flg_Inproc : FVT_lib/outp/OverrideAndLimit  SystemSampleTime=-1  VariantActivationTime=update diagram  Latency=0  AutoFrameSizeCalculation=off
      link override Signal_Limit/_maxval: Value=KOUTP_FrActvDmpDisabReq_flg_maxval
      link override Signal_Limit/_minval: Value=KOUTP_FrActvDmpDisabReq_flg_minval
      link override Signal_Override/_ovrdflg: Value=KOUTP_FrActvDmpDisabReq_flg_ovrdflg
      link override Signal_Override/_ovrdval: Value=KOUTP_FrActvDmpDisabReq_flg_ovrdval
  VTQD_FrEDUActTq_Nm_Inproc : FVT_lib/outp/OverrideAndLimit  SystemSampleTime=-1  VariantActivationTime=update diagram  Latency=0  AutoFrameSizeCalculation=off
      link override Signal_Limit/_maxval: Value=KOUTP_FrEDUActTq_Nm_maxval
      link override Signal_Limit/_minval: Value=KOUTP_FrEDUActTq_Nm_minval
      link override Signal_Override/_ovrdflg: Value=KOUTP_FrEDUActTq_Nm_ovrdflg
      link override Signal_Override/_ovrdval: Value=KOUTP_FrEDUActTq_Nm_ovrdval
  VTQD_FrEDUAvailBrkRgnTqV_flg_Inproc : FVT_lib/outp/OverrideAndLimit  SystemSampleTime=-1  VariantActivationTime=update diagram  Latency=0  AutoFrameSizeCalculation=off
      link override Signal_Limit/_maxval: Value=KOUTP_FrEDUAvailBrkRgnTqV_flg_maxval
      link override Signal_Limit/_minval: Value=KOUTP_FrEDUAvailBrkRgnTqV_flg_minval
      link override Signal_Override/_ovrdflg: Value=KOUTP_FrEDUAvailBrkRgnTqV_flg_ovrdflg
      link override Signal_Override/_ovrdval: Value=KOUTP_FrEDUAvailBrkRgnTqV_flg_ovrdval
  VTQD_FrEDUAvailBrkRgnTq_Nm_Inproc : FVT_lib/outp/OverrideAndLimit  SystemSampleTime=-1  VariantActivationTime=update diagram  Latency=0  AutoFrameSizeCalculation=off
      link override Signal_Limit/_maxval: Value=KOUTP_FrEDUAvailBrkRgnTq_Nm_maxval
      link override Signal_Limit/_minval: Value=KOUTP_FrEDUAvailBrkRgnTq_Nm_minval
      link override Signal_Override/_ovrdflg: Value=KOUTP_FrEDUAvailBrkRgnTq_Nm_ovrdflg
      link override Signal_Override/_ovrdval: Value=KOUTP_FrEDUAvailBrkRgnTq_Nm_ovrdval
  VTQD_FrEDURolRgnTq_Nm_Inproc : FVT_lib/outp/OverrideAndLimit  SystemSampleTime=-1  VariantActivationTime=update diagram  Latency=0  AutoFrameSizeCalculation=off
      link override Signal_Limit/_maxval: Value=KOUTP_FrEDURolRgnTq_Nm_maxval
      link override Signal_Limit/_minval: Value=KOUTP_FrEDURolRgnTq_Nm_minval
      link override Signal_Override/_ovrdflg: Value=KOUTP_FrEDURolRgnTq_Nm_ovrdflg
      link override Signal_Override/_ovrdval: Value=KOUTP_FrEDURolRgnTq_Nm_ovrdval
  VTQD_FrEDUSpdValid_flg_Inproc : FVT_lib/outp/OverrideAndLimit  SystemSampleTime=-1  VariantActivationTime=update diagram  Latency=0  AutoFrameSizeCalculation=off
      link override Signal_Limit/_maxval: Value=KOUTP_FrEDUSpdValid_flg_maxval
      link override Signal_Limit/_minval: Value=KOUTP_FrEDUSpdValid_flg_minval
      link override Signal_Override/_ovrdflg: Value=KOUTP_FrEDUSpdValid_flg_ovrdflg
      link override Signal_Override/_ovrdval: Value=KOUTP_FrEDUSpdValid_flg_ovrdval
  VTQD_FrEDUSpd_rpm_Inproc : FVT_lib/outp/OverrideAndLimit  SystemSampleTime=-1  VariantActivationTime=update diagram  Latency=0  AutoFrameSizeCalculation=off
      link override Signal_Limit/_maxval: Value=KOUTP_FrEDUSpd_rpm_maxval
      link override Signal_Limit/_minval: Value=KOUTP_FrEDUSpd_rpm_minval
      link override Signal_Override/_ovrdflg: Value=KOUTP_FrEDUSpd_rpm_ovrdflg
      link override Signal_Override/_ovrdval: Value=KOUTP_FrEDUSpd_rpm_ovrdval
  VTQD_FrIdcMax_A_Inproc : FVT_lib/outp/OverrideAndLimit  SystemSampleTime=-1  VariantActivationTime=update diagram  Latency=0  AutoFrameSizeCalculation=off
      link override Signal_Limit/_maxval: Value=KOUTP_FrIdcMax_A_maxval
      link override Signal_Limit/_minval: Value=KOUTP_FrIdcMax_A_minval
      link override Signal_Override/_ovrdflg: Value=KOUTP_FrIdcMax_A_ovrdflg
      link override Signal_Override/_ovrdval: Value=KOUTP_FrIdcMax_A_ovrdval
  VTQD_FrIdcMin_A_Inproc : FVT_lib/outp/OverrideAndLimit  SystemSampleTime=-1  VariantActivationTime=update diagram  Latency=0  AutoFrameSizeCalculation=off
      link override Signal_Limit/_maxval: Value=KOUTP_FrIdcMin_A_maxval
      link override Signal_Limit/_minval: Value=KOUTP_FrIdcMin_A_minval
      link override Signal_Override/_ovrdflg: Value=KOUTP_FrIdcMin_A_ovrdflg
      link override Signal_Override/_ovrdval: Value=KOUTP_FrIdcMin_A_ovrdval
  VTQD_FrRgnDecrSta_flg_Inproc : FVT_lib/outp/OverrideAndLimit  SystemSampleTime=-1  VariantActivationTime=update diagram  Latency=0  AutoFrameSizeCalculation=off
      link override Signal_Limit/_maxval: Value=KOUTP_FrRgnDecrSta_flg_maxval
      link override Signal_Limit/_minval: Value=KOUTP_FrRgnDecrSta_flg_minval
      link override Signal_Override/_ovrdflg: Value=KOUTP_FrRgnDecrSta_flg_ovrdflg
      link override Signal_Override/_ovrdval: Value=KOUTP_FrRgnDecrSta_flg_ovrdval
  VTQD_FrRgnPermSta_flg_Inproc : FVT_lib/outp/OverrideAndLimit  SystemSampleTime=-1  VariantActivationTime=update diagram  Latency=0  AutoFrameSizeCalculation=off
      link override Signal_Limit/_maxval: Value=KOUTP_FrRgnPermSta_flg_maxval
      link override Signal_Limit/_minval: Value=KOUTP_FrRgnPermSta_flg_minval
      link override Signal_Override/_ovrdflg: Value=KOUTP_FrRgnPermSta_flg_ovrdflg
      link override Signal_Override/_ovrdval: Value=KOUTP_FrRgnPermSta_flg_ovrdval
  VTQD_FrUdcMax_V_Inproc : FVT_lib/outp/OverrideAndLimit  SystemSampleTime=-1  VariantActivationTime=update diagram  Latency=0  AutoFrameSizeCalculation=off
      link override Signal_Limit/_maxval: Value=KOUTP_FrUdcMax_V_maxval
      link override Signal_Limit/_minval: Value=KOUTP_FrUdcMax_V_minval
      link override Signal_Override/_ovrdflg: Value=KOUTP_FrUdcMax_V_ovrdflg
      link override Signal_Override/_ovrdval: Value=KOUTP_FrUdcMax_V_ovrdval
  VTQD_FrUdcMin_V_Inproc : FVT_lib/outp/OverrideAndLimit  SystemSampleTime=-1  VariantActivationTime=update diagram  Latency=0  AutoFrameSizeCalculation=off
      link override Signal_Limit/_maxval: Value=KOUTP_FrUdcMin_V_maxval
      link override Signal_Limit/_minval: Value=KOUTP_FrUdcMin_V_minval
      link override Signal_Override/_ovrdflg: Value=KOUTP_FrUdcMin_V_ovrdflg
      link override Signal_Override/_ovrdval: Value=KOUTP_FrUdcMin_V_ovrdval
  VTQD_IVIPwrLockSta_enum_Inproc : FVT_lib/outp/OverrideAndLimit  SystemSampleTime=-1  VariantActivationTime=update diagram  Latency=0  AutoFrameSizeCalculation=off
      link override Signal_Limit/_maxval: Value=KOUTP_IVIPwrLockSta_enum_maxval
      link override Signal_Limit/_minval: Value=KOUTP_IVIPwrLockSta_enum_minval
      link override Signal_Override/_ovrdflg: Value=KOUTP_IVIPwrLockSta_enum_ovrdflg
      link override Signal_Override/_ovrdval: Value=KOUTP_IVIPwrLockSta_enum_ovrdval
  VTQD_OPDHoldLamp_flg_Inproc : FVT_lib/outp/OverrideAndLimit  SystemSampleTime=-1  VariantActivationTime=update diagram  Latency=0  AutoFrameSizeCalculation=off
      link override Signal_Limit/_maxval: Value=KOUTP_OPDHoldLamp_flg_maxval
      link override Signal_Limit/_minval: Value=KOUTP_OPDHoldLamp_flg_minval
      link override Signal_Override/_ovrdflg: Value=KOUTP_OPDHoldLamp_flg_ovrdflg
      link override Signal_Override/_ovrdval: Value=KOUTP_OPDHoldLamp_flg_ovrdval
  VTQD_PButtonSta_enum_Inproc : FVT_lib/outp/OverrideAndLimit  SystemSampleTime=-1  VariantActivationTime=update diagram  Latency=0  AutoFrameSizeCalculation=off
      link override Signal_Limit/_maxval: Value=KOUTP_PButtonSta_enum_maxval
      link override Signal_Limit/_minval: Value=KOUTP_PButtonSta_enum_minval
      link override Signal_Override/_ovrdflg: Value=KOUTP_PButtonSta_enum_ovrdflg
      link override Signal_Override/_ovrdval: Value=KOUTP_PButtonSta_enum_ovrdval
  VTQD_PTCSPermSta_flg_Inproc : FVT_lib/outp/OverrideAndLimit  SystemSampleTime=-1  VariantActivationTime=update diagram  Latency=0  AutoFrameSizeCalculation=off
      link override Signal_Limit/_maxval: Value=KOUTP_PTCSPermSta_flg_maxval
      link override Signal_Limit/_minval: Value=KOUTP_PTCSPermSta_flg_minval
      link override Signal_Override/_ovrdflg: Value=KOUTP_PTCSPermSta_flg_ovrdflg
      link override Signal_Override/_ovrdval: Value=KOUTP_PTCSPermSta_flg_ovrdval
  VTQD_ParkRequest_flg_Inproc : FVT_lib/outp/OverrideAndLimit  SystemSampleTime=-1  VariantActivationTime=update diagram  Latency=0  AutoFrameSizeCalculation=off
      link override Signal_Limit/_maxval: Value=KOUTP_ParkRequest_flg_maxval
      link override Signal_Limit/_minval: Value=KOUTP_ParkRequest_flg_minval
      link override Signal_Override/_ovrdflg: Value=KOUTP_ParkRequest_flg_ovrdflg
      link override Signal_Override/_ovrdval: Value=KOUTP_ParkRequest_flg_ovrdval
  VTQD_ReBrakeLPReq_flg_Inproc : FVT_lib/outp/OverrideAndLimit  SystemSampleTime=-1  VariantActivationTime=update diagram  Latency=0  AutoFrameSizeCalculation=off
      link override Signal_Limit/_maxval: Value=KOUTP_ReBrakeLPReq_flg_maxval
      link override Signal_Limit/_minval: Value=KOUTP_ReBrakeLPReq_flg_minval
      link override Signal_Override/_ovrdflg: Value=KOUTP_ReBrakeLPReq_flg_ovrdflg
      link override Signal_Override/_ovrdval: Value=KOUTP_ReBrakeLPReq_flg_ovrdval
  VTQD_RegenLimIndSta_flg_Inproc : FVT_lib/outp/OverrideAndLimit  SystemSampleTime=-1  VariantActivationTime=update diagram  Latency=0  AutoFrameSizeCalculation=off
      link override Signal_Limit/_maxval: Value=KOUTP_RegenLimIndSta_flg_maxval
      link override Signal_Limit/_minval: Value=KOUTP_RegenLimIndSta_flg_minval
      link override Signal_Override/_ovrdflg: Value=KOUTP_RegenLimIndSta_flg_ovrdflg
      link override Signal_Override/_ovrdval: Value=KOUTP_RegenLimIndSta_flg_ovrdval
  VTQD_RgnAbnorSta_flg_Inproc : FVT_lib/outp/OverrideAndLimit  SystemSampleTime=-1  VariantActivationTime=update diagram  Latency=0  AutoFrameSizeCalculation=off
      link override Signal_Limit/_maxval: Value=KOUTP_RgnAbnorSta_flg_maxval
      link override Signal_Limit/_minval: Value=KOUTP_RgnAbnorSta_flg_minval
      link override Signal_Override/_ovrdflg: Value=KOUTP_RgnAbnorSta_flg_ovrdflg
      link override Signal_Override/_ovrdval: Value=KOUTP_RgnAbnorSta_flg_ovrdval
  VTQD_RrActvDmpDisabReq_flg_Inproc : FVT_lib/outp/OverrideAndLimit  SystemSampleTime=-1  VariantActivationTime=update diagram  Latency=0  AutoFrameSizeCalculation=off
      link override Signal_Limit/_maxval: Value=KOUTP_RrActvDmpDisabReq_flg_maxval
      link override Signal_Limit/_minval: Value=KOUTP_RrActvDmpDisabReq_flg_minval
      link override Signal_Override/_ovrdflg: Value=KOUTP_RrActvDmpDisabReq_flg_ovrdflg
      link override Signal_Override/_ovrdval: Value=KOUTP_RrActvDmpDisabReq_flg_ovrdval
  VTQD_RrEDUActTq_Nm_Inproc : FVT_lib/outp/OverrideAndLimit  SystemSampleTime=-1  VariantActivationTime=update diagram  Latency=0  AutoFrameSizeCalculation=off
      link override Signal_Limit/_maxval: Value=KOUTP_RrEDUActTq_Nm_maxval
      link override Signal_Limit/_minval: Value=KOUTP_RrEDUActTq_Nm_minval
      link override Signal_Override/_ovrdflg: Value=KOUTP_RrEDUActTq_Nm_ovrdflg
      link override Signal_Override/_ovrdval: Value=KOUTP_RrEDUActTq_Nm_ovrdval
  VTQD_RrEDUAvailBrkRgnTqV_flg_Inproc : FVT_lib/outp/OverrideAndLimit  SystemSampleTime=-1  VariantActivationTime=update diagram  Latency=0  AutoFrameSizeCalculation=off
      link override Signal_Limit/_maxval: Value=KOUTP_RrEDUAvailBrkRgnTqV_flg_maxval
      link override Signal_Limit/_minval: Value=KOUTP_RrEDUAvailBrkRgnTqV_flg_minval
      link override Signal_Override/_ovrdflg: Value=KOUTP_RrEDUAvailBrkRgnTqV_flg_ovrdflg
      link override Signal_Override/_ovrdval: Value=KOUTP_RrEDUAvailBrkRgnTqV_flg_ovrdval
  VTQD_RrEDUAvailBrkRgnTq_Nm_Inproc : FVT_lib/outp/OverrideAndLimit  SystemSampleTime=-1  VariantActivationTime=update diagram  Latency=0  AutoFrameSizeCalculation=off
      link override Signal_Limit/_maxval: Value=KOUTP_RrEDUAvailBrkRgnTq_Nm_maxval
      link override Signal_Limit/_minval: Value=KOUTP_RrEDUAvailBrkRgnTq_Nm_minval
      link override Signal_Override/_ovrdflg: Value=KOUTP_RrEDUAvailBrkRgnTq_Nm_ovrdflg
      link override Signal_Override/_ovrdval: Value=KOUTP_RrEDUAvailBrkRgnTq_Nm_ovrdval
  VTQD_RrEDURolRgnTq_Nm_Inproc : FVT_lib/outp/OverrideAndLimit  SystemSampleTime=-1  VariantActivationTime=update diagram  Latency=0  AutoFrameSizeCalculation=off
      link override Signal_Limit/_maxval: Value=KOUTP_RrEDURolRgnTq_Nm_maxval
      link override Signal_Limit/_minval: Value=KOUTP_RrEDURolRgnTq_Nm_minval
      link override Signal_Override/_ovrdflg: Value=KOUTP_RrEDURolRgnTq_Nm_ovrdflg
      link override Signal_Override/_ovrdval: Value=KOUTP_RrEDURolRgnTq_Nm_ovrdval
  VTQD_RrEDUSpdValid_flg_Inproc : FVT_lib/outp/OverrideAndLimit  SystemSampleTime=-1  VariantActivationTime=update diagram  Latency=0  AutoFrameSizeCalculation=off
      link override Signal_Limit/_maxval: Value=KOUTP_RrEDUSpdValid_flg_maxval
      link override Signal_Limit/_minval: Value=KOUTP_RrEDUSpdValid_flg_minval
      link override Signal_Override/_ovrdflg: Value=KOUTP_RrEDUSpdValid_flg_ovrdflg
      link override Signal_Override/_ovrdval: Value=KOUTP_RrEDUSpdValid_flg_ovrdval
  VTQD_RrEDUSpd_rpm_Inproc : FVT_lib/outp/OverrideAndLimit  SystemSampleTime=-1  VariantActivationTime=update diagram  Latency=0  AutoFrameSizeCalculation=off
      link override Signal_Limit/_maxval: Value=KOUTP_RrEDUSpd_rpm_maxval
      link override Signal_Limit/_minval: Value=KOUTP_RrEDUSpd_rpm_minval
      link override Signal_Override/_ovrdflg: Value=KOUTP_RrEDUSpd_rpm_ovrdflg
      link override Signal_Override/_ovrdval: Value=KOUTP_RrEDUSpd_rpm_ovrdval
  VTQD_RrIdcMax_A_Inproc : FVT_lib/outp/OverrideAndLimit  SystemSampleTime=-1  VariantActivationTime=update diagram  Latency=0  AutoFrameSizeCalculation=off
      link override Signal_Limit/_maxval: Value=KOUTP_RrIdcMax_A_maxval
      link override Signal_Limit/_minval: Value=KOUTP_RrIdcMax_A_minval
      link override Signal_Override/_ovrdflg: Value=KOUTP_RrIdcMax_A_ovrdflg
      link override Signal_Override/_ovrdval: Value=KOUTP_RrIdcMax_A_ovrdval
  VTQD_RrIdcMin_A_Inproc : FVT_lib/outp/OverrideAndLimit  SystemSampleTime=-1  VariantActivationTime=update diagram  Latency=0  AutoFrameSizeCalculation=off
      link override Signal_Limit/_maxval: Value=KOUTP_RrIdcMin_A_maxval
      link override Signal_Limit/_minval: Value=KOUTP_RrIdcMin_A_minval
      link override Signal_Override/_ovrdflg: Value=KOUTP_RrIdcMin_A_ovrdflg
      link override Signal_Override/_ovrdval: Value=KOUTP_RrIdcMin_A_ovrdval
  VTQD_RrRgnDecrSta_flg_Inproc : FVT_lib/outp/OverrideAndLimit  SystemSampleTime=-1  VariantActivationTime=update diagram  Latency=0  AutoFrameSizeCalculation=off
      link override Signal_Limit/_maxval: Value=KOUTP_RrRgnDecrSta_flg_maxval
      link override Signal_Limit/_minval: Value=KOUTP_RrRgnDecrSta_flg_minval
      link override Signal_Override/_ovrdflg: Value=KOUTP_RrRgnDecrSta_flg_ovrdflg
      link override Signal_Override/_ovrdval: Value=KOUTP_RrRgnDecrSta_flg_ovrdval
  VTQD_RrRgnPermSta_flg_Inproc : FVT_lib/outp/OverrideAndLimit  SystemSampleTime=-1  VariantActivationTime=update diagram  Latency=0  AutoFrameSizeCalculation=off
      link override Signal_Limit/_maxval: Value=KOUTP_RrRgnPermSta_flg_maxval
      link override Signal_Limit/_minval: Value=KOUTP_RrRgnPermSta_flg_minval
      link override Signal_Override/_ovrdflg: Value=KOUTP_RrRgnPermSta_flg_ovrdflg
      link override Signal_Override/_ovrdval: Value=KOUTP_RrRgnPermSta_flg_ovrdval
  VTQD_RrUdcMax_V_Inproc : FVT_lib/outp/OverrideAndLimit  SystemSampleTime=-1  VariantActivationTime=update diagram  Latency=0  AutoFrameSizeCalculation=off
      link override Signal_Limit/_maxval: Value=KOUTP_RrUdcMax_V_maxval
      link override Signal_Limit/_minval: Value=KOUTP_RrUdcMax_V_minval
      link override Signal_Override/_ovrdflg: Value=KOUTP_RrUdcMax_V_ovrdflg
      link override Signal_Override/_ovrdval: Value=KOUTP_RrUdcMax_V_ovrdval
  VTQD_RrUdcMin_V_Inproc : FVT_lib/outp/OverrideAndLimit  SystemSampleTime=-1  VariantActivationTime=update diagram  Latency=0  AutoFrameSizeCalculation=off
      link override Signal_Limit/_maxval: Value=KOUTP_RrUdcMin_V_maxval
      link override Signal_Limit/_minval: Value=KOUTP_RrUdcMin_V_minval
      link override Signal_Override/_ovrdflg: Value=KOUTP_RrUdcMin_V_ovrdflg
      link override Signal_Override/_ovrdval: Value=KOUTP_RrUdcMin_V_ovrdval
  VTQD_SaveRegenMode_enum_Inproc : FVT_lib/outp/OverrideAndLimit  SystemSampleTime=-1  VariantActivationTime=update diagram  Latency=0  AutoFrameSizeCalculation=off
      link override Signal_Limit/_maxval: Value=KOUTP_SaveRegenMode_enum_maxval
      link override Signal_Limit/_minval: Value=KOUTP_SaveRegenMode_enum_minval
      link override Signal_Override/_ovrdflg: Value=KOUTP_SaveRegenMode_enum_ovrdflg
      link override Signal_Override/_ovrdval: Value=KOUTP_SaveRegenMode_enum_ovrdval
  VTQD_SetSpdLimWarn_flg_Inproc : FVT_lib/outp/OverrideAndLimit  SystemSampleTime=-1  VariantActivationTime=update diagram  Latency=0  AutoFrameSizeCalculation=off
      link override Signal_Limit/_maxval: Value=KOUTP_SetSpdLimWarn_flg_maxval
      link override Signal_Limit/_minval: Value=KOUTP_SetSpdLimWarn_flg_minval
      link override Signal_Override/_ovrdflg: Value=KOUTP_SetSpdLimWarn_flg_ovrdflg
      link override Signal_Override/_ovrdval: Value=KOUTP_SetSpdLimWarn_flg_ovrdval
  VTQD_SetSpd_kph_Inproc : FVT_lib/outp/OverrideAndLimit  SystemSampleTime=-1  VariantActivationTime=update diagram  Latency=0  AutoFrameSizeCalculation=off
      link override Signal_Limit/_maxval: Value=KOUTP_SetSpd_kph_maxval
      link override Signal_Limit/_minval: Value=KOUTP_SetSpd_kph_minval
      link override Signal_Override/_ovrdflg: Value=KOUTP_SetSpd_kph_ovrdflg
      link override Signal_Override/_ovrdval: Value=KOUTP_SetSpd_kph_ovrdval
  VTQD_ShiftGearPosn_enum_Inproc : FVT_lib/outp/OverrideAndLimit  SystemSampleTime=-1  VariantActivationTime=update diagram  Latency=0  AutoFrameSizeCalculation=off
      link override Signal_Limit/_maxval: Value=KOUTP_ShiftGearPosn_enum_maxval
      link override Signal_Limit/_minval: Value=KOUTP_ShiftGearPosn_enum_minval
      link override Signal_Override/_ovrdflg: Value=KOUTP_ShiftGearPosn_enum_ovrdflg
      link override Signal_Override/_ovrdval: Value=KOUTP_ShiftGearPosn_enum_ovrdval
  VTQD_SpdCtrlMode_enum_Inproc : FVT_lib/outp/OverrideAndLimit  SystemSampleTime=-1  VariantActivationTime=update diagram  Latency=0  AutoFrameSizeCalculation=off
      link override Signal_Limit/_maxval: Value=KOUTP_SpdCtrlMode_enum_maxval
      link override Signal_Limit/_minval: Value=KOUTP_SpdCtrlMode_enum_minval
      link override Signal_Override/_ovrdflg: Value=KOUTP_SpdCtrlMode_enum_ovrdflg
      link override Signal_Override/_ovrdval: Value=KOUTP_SpdCtrlMode_enum_ovrdval
  VTQD_SpdCtrlSta_flg_Inproc : FVT_lib/outp/OverrideAndLimit  SystemSampleTime=-1  VariantActivationTime=update diagram  Latency=0  AutoFrameSizeCalculation=off
      link override Signal_Limit/_maxval: Value=KOUTP_SpdCtrlSta_flg_maxval
      link override Signal_Limit/_minval: Value=KOUTP_SpdCtrlSta_flg_minval
      link override Signal_Override/_ovrdflg: Value=KOUTP_SpdCtrlSta_flg_ovrdflg
      link override Signal_Override/_ovrdval: Value=KOUTP_SpdCtrlSta_flg_ovrdval
  VTQD_TqSourceFr_enum_Inproc : FVT_lib/outp/OverrideAndLimit  SystemSampleTime=-1  VariantActivationTime=update diagram  Latency=0  AutoFrameSizeCalculation=off
      link override Signal_Limit/_maxval: Value=KOUTP_TqSourceFr_enum_maxval
      link override Signal_Limit/_minval: Value=KOUTP_TqSourceFr_enum_minval
      link override Signal_Override/_ovrdflg: Value=KOUTP_TqSourceFr_enum_ovrdflg
      link override Signal_Override/_ovrdval: Value=KOUTP_TqSourceFr_enum_ovrdval
  VTQD_TqSourceRr_enum_Inproc : FVT_lib/outp/OverrideAndLimit  SystemSampleTime=-1  VariantActivationTime=update diagram  Latency=0  AutoFrameSizeCalculation=off
      link override Signal_Limit/_maxval: Value=KOUTP_TqSourceRr_enum_maxval
      link override Signal_Limit/_minval: Value=KOUTP_TqSourceRr_enum_minval
      link override Signal_Override/_ovrdflg: Value=KOUTP_TqSourceRr_enum_ovrdflg
      link override Signal_Override/_ovrdval: Value=KOUTP_TqSourceRr_enum_ovrdval
  VTQD_VehActSpd_kph_Inproc : FVT_lib/outp/OverrideAndLimit  SystemSampleTime=-1  VariantActivationTime=update diagram  Latency=0  AutoFrameSizeCalculation=off
      link override Signal_Limit/_maxval: Value=KOUTP_VehActSpd_kph_maxval
      link override Signal_Limit/_minval: Value=KOUTP_VehActSpd_kph_minval
      link override Signal_Override/_ovrdflg: Value=KOUTP_VehActSpd_kph_ovrdflg
      link override Signal_Override/_ovrdval: Value=KOUTP_VehActSpd_kph_ovrdval
  VTQR_FrTMTqReq_Nm_Inproc : FVT_lib/outp/OverrideAndLimit  SystemSampleTime=-1  VariantActivationTime=update diagram  Latency=0  AutoFrameSizeCalculation=off
      link override Signal_Limit/_maxval: Value=KOUTP_FrTMTqReq_Nm_maxval
      link override Signal_Limit/_minval: Value=KOUTP_FrTMTqReq_Nm_minval
      link override Signal_Override/_ovrdflg: Value=KOUTP_FrTMTqReq_Nm_ovrdflg
      link override Signal_Override/_ovrdval: Value=KOUTP_FrTMTqReq_Nm_ovrdval
  VTQR_RrTMTqReq_Nm_Inproc : FVT_lib/outp/OverrideAndLimit  SystemSampleTime=-1  VariantActivationTime=update diagram  Latency=0  AutoFrameSizeCalculation=off
      link override Signal_Limit/_maxval: Value=KOUTP_RrTMTqReq_Nm_maxval
      link override Signal_Limit/_minval: Value=KOUTP_RrTMTqReq_Nm_minval
      link override Signal_Override/_ovrdflg: Value=KOUTP_RrTMTqReq_Nm_ovrdflg
      link override Signal_Override/_ovrdval: Value=KOUTP_RrTMTqReq_Nm_ovrdval
  VV2L_HVPO120VGrpALDSt_enum_Inproc : FVT_lib/outp/OverrideAndLimit  SystemSampleTime=-1  VariantActivationTime=update diagram  Latency=0  AutoFrameSizeCalculation=off
      link override Signal_Limit/_maxval: Value=KOUTP_HVPO120VGrpALDSt_enum_maxval
      link override Signal_Limit/_minval: Value=KOUTP_HVPO120VGrpALDSt_enum_minval
      link override Signal_Override/_ovrdflg: Value=KOUTP_HVPO120VGrpALDSt_enum_ovrdflg
      link override Signal_Override/_ovrdval: Value=KOUTP_HVPO120VGrpALDSt_enum_ovrdval
  VV2L_HVPO120VGrpBLDSt_enum_Inproc : FVT_lib/outp/OverrideAndLimit  SystemSampleTime=-1  VariantActivationTime=update diagram  Latency=0  AutoFrameSizeCalculation=off
      link override Signal_Limit/_maxval: Value=KOUTP_HVPO120VGrpBLDSt_enum_maxval
      link override Signal_Limit/_minval: Value=KOUTP_HVPO120VGrpBLDSt_enum_minval
      link override Signal_Override/_ovrdflg: Value=KOUTP_HVPO120VGrpBLDSt_enum_ovrdflg
      link override Signal_Override/_ovrdval: Value=KOUTP_HVPO120VGrpBLDSt_enum_ovrdval
  VV2L_ReqOBCExtrV2LEna_enum_Inproc : FVT_lib/outp/OverrideAndLimit  SystemSampleTime=-1  VariantActivationTime=update diagram  Latency=0  AutoFrameSizeCalculation=off
      link override Signal_Limit/_maxval: Value=KOUTP_ReqOBCExtrV2LEna_enum_maxval
      link override Signal_Limit/_minval: Value=KOUTP_ReqOBCExtrV2LEna_enum_minval
      link override Signal_Override/_ovrdflg: Value=KOUTP_ReqOBCExtrV2LEna_enum_ovrdflg
      link override Signal_Override/_ovrdval: Value=KOUTP_ReqOBCExtrV2LEna_enum_ovrdval
  VV2L_ReqOBCIntrV2LEna_enum_Inproc : FVT_lib/outp/OverrideAndLimit  SystemSampleTime=-1  VariantActivationTime=update diagram  Latency=0  AutoFrameSizeCalculation=off
      link override Signal_Limit/_maxval: Value=KOUTP_ReqOBCIntrV2LEna_enum_maxval
      link override Signal_Limit/_minval: Value=KOUTP_ReqOBCIntrV2LEna_enum_minval
      link override Signal_Override/_ovrdflg: Value=KOUTP_ReqOBCIntrV2LEna_enum_ovrdflg
      link override Signal_Override/_ovrdval: Value=KOUTP_ReqOBCIntrV2LEna_enum_ovrdval
  VV2L_ReqOBCV2LEna_enum_Inproc : FVT_lib/outp/OverrideAndLimit  SystemSampleTime=-1  VariantActivationTime=update diagram  Latency=0  AutoFrameSizeCalculation=off
      link override Signal_Limit/_maxval: Value=KOUTP_ReqOBCV2LEna_enum_maxval
      link override Signal_Limit/_minval: Value=KOUTP_ReqOBCV2LEna_enum_minval
      link override Signal_Override/_ovrdflg: Value=KOUTP_ReqOBCV2LEna_enum_ovrdflg
      link override Signal_Override/_ovrdval: Value=KOUTP_ReqOBCV2LEna_enum_ovrdval
  VV2L_ReqV2LIVIDisChrg_enum_Inproc : FVT_lib/outp/OverrideAndLimit  SystemSampleTime=-1  VariantActivationTime=update diagram  Latency=0  AutoFrameSizeCalculation=off
      link override Signal_Limit/_maxval: Value=KOUTP_ReqV2LIVIDisChrg_enum_maxval
      link override Signal_Limit/_minval: Value=KOUTP_ReqV2LIVIDisChrg_enum_minval
      link override Signal_Override/_ovrdflg: Value=KOUTP_ReqV2LIVIDisChrg_enum_ovrdflg
      link override Signal_Override/_ovrdval: Value=KOUTP_ReqV2LIVIDisChrg_enum_ovrdval
  VV2L_ReqV2LIVIPopup_enum_Inproc : FVT_lib/outp/OverrideAndLimit  SystemSampleTime=-1  VariantActivationTime=update diagram  Latency=0  AutoFrameSizeCalculation=off
      link override Signal_Limit/_maxval: Value=KOUTP_ReqV2LIVIPopup_enum_maxval
      link override Signal_Limit/_minval: Value=KOUTP_ReqV2LIVIPopup_enum_minval
      link override Signal_Override/_ovrdflg: Value=KOUTP_ReqV2LIVIPopup_enum_ovrdflg
      link override Signal_Override/_ovrdval: Value=KOUTP_ReqV2LIVIPopup_enum_ovrdval
  VVMC_ACCComfortBandLower_mps2_Inproc : FVT_lib/outp/OverrideAndLimit  SystemSampleTime=-1  VariantActivationTime=update diagram  Latency=0  AutoFrameSizeCalculation=off
      link override Signal_Limit/_maxval: Value=KOUTP_ACCComfortBandLower_mps2_maxval
      link override Signal_Limit/_minval: Value=KOUTP_ACCComfortBandLower_mps2_minval
      link override Signal_Override/_ovrdflg: Value=KOUTP_ACCComfortBandLower_mps2_ovrdflg
      link override Signal_Override/_ovrdval: Value=KOUTP_ACCComfortBandLower_mps2_ovrdval
  VVMC_ACCComfortBandUpper_mps2_Inproc : FVT_lib/outp/OverrideAndLimit  SystemSampleTime=-1  VariantActivationTime=update diagram  Latency=0  AutoFrameSizeCalculation=off
      link override Signal_Limit/_maxval: Value=KOUTP_ACCComfortBandUpper_mps2_maxval
      link override Signal_Limit/_minval: Value=KOUTP_ACCComfortBandUpper_mps2_minval
      link override Signal_Override/_ovrdflg: Value=KOUTP_ACCComfortBandUpper_mps2_ovrdflg
      link override Signal_Override/_ovrdval: Value=KOUTP_ACCComfortBandUpper_mps2_ovrdval
  VVMC_ACCCtrlAvail_flg_Inproc : FVT_lib/outp/OverrideAndLimit  SystemSampleTime=-1  VariantActivationTime=update diagram  Latency=0  AutoFrameSizeCalculation=off
      link override Signal_Limit/_maxval: Value=KOUTP_ACCCtrlAvail_flg_maxval
      link override Signal_Limit/_minval: Value=KOUTP_ACCCtrlAvail_flg_minval
      link override Signal_Override/_ovrdflg: Value=KOUTP_ACCCtrlAvail_flg_ovrdflg
      link override Signal_Override/_ovrdval: Value=KOUTP_ACCCtrlAvail_flg_ovrdval
  VVMC_ACCJerkLowerLimit_mps3_Inproc : FVT_lib/outp/OverrideAndLimit  SystemSampleTime=-1  VariantActivationTime=update diagram  Latency=0  AutoFrameSizeCalculation=off
      link override Signal_Limit/_maxval: Value=KOUTP_ACCJerkLowerLimit_mps3_maxval
      link override Signal_Limit/_minval: Value=KOUTP_ACCJerkLowerLimit_mps3_minval
      link override Signal_Override/_ovrdflg: Value=KOUTP_ACCJerkLowerLimit_mps3_ovrdflg
      link override Signal_Override/_ovrdval: Value=KOUTP_ACCJerkLowerLimit_mps3_ovrdval
  VVMC_ACCJerkUpperLimit_mps3_Inproc : FVT_lib/outp/OverrideAndLimit  SystemSampleTime=-1  VariantActivationTime=update diagram  Latency=0  AutoFrameSizeCalculation=off
      link override Signal_Limit/_maxval: Value=KOUTP_ACCJerkUpperLimit_mps3_maxval
      link override Signal_Limit/_minval: Value=KOUTP_ACCJerkUpperLimit_mps3_minval
      link override Signal_Override/_ovrdflg: Value=KOUTP_ACCJerkUpperLimit_mps3_ovrdflg
      link override Signal_Override/_ovrdval: Value=KOUTP_ACCJerkUpperLimit_mps3_ovrdval
  VVMC_ACCObjDist_m_Inproc : FVT_lib/outp/OverrideAndLimit  SystemSampleTime=-1  VariantActivationTime=update diagram  Latency=0  AutoFrameSizeCalculation=off
      link override Signal_Limit/_maxval: Value=KOUTP_ACCObjDist_m_maxval
      link override Signal_Limit/_minval: Value=KOUTP_ACCObjDist_m_minval
      link override Signal_Override/_ovrdflg: Value=KOUTP_ACCObjDist_m_ovrdflg
      link override Signal_Override/_ovrdval: Value=KOUTP_ACCObjDist_m_ovrdval
  VVMC_ACCObjDstLvl_enum_Inproc : FVT_lib/outp/OverrideAndLimit  SystemSampleTime=-1  VariantActivationTime=update diagram  Latency=0  AutoFrameSizeCalculation=off
      link override Signal_Limit/_maxval: Value=KOUTP_ACCObjDstLvl_enum_maxval
      link override Signal_Limit/_minval: Value=KOUTP_ACCObjDstLvl_enum_minval
      link override Signal_Override/_ovrdflg: Value=KOUTP_ACCObjDstLvl_enum_ovrdflg
      link override Signal_Override/_ovrdval: Value=KOUTP_ACCObjDstLvl_enum_ovrdval
  VVMC_ACCObjRelSpd_mps_Inproc : FVT_lib/outp/OverrideAndLimit  SystemSampleTime=-1  VariantActivationTime=update diagram  Latency=0  AutoFrameSizeCalculation=off
      link override Signal_Limit/_maxval: Value=KOUTP_ACCObjRelSpd_mps_maxval
      link override Signal_Limit/_minval: Value=KOUTP_ACCObjRelSpd_mps_minval
      link override Signal_Override/_ovrdflg: Value=KOUTP_ACCObjRelSpd_mps_ovrdflg
      link override Signal_Override/_ovrdval: Value=KOUTP_ACCObjRelSpd_mps_ovrdval
  VVMC_ACCPedalOvrd_flg_Inproc : FVT_lib/outp/OverrideAndLimit  SystemSampleTime=-1  VariantActivationTime=update diagram  Latency=0  AutoFrameSizeCalculation=off
      link override Signal_Limit/_maxval: Value=KOUTP_ACCPedalOvrd_flg_maxval
      link override Signal_Limit/_minval: Value=KOUTP_ACCPedalOvrd_flg_minval
      link override Signal_Override/_ovrdflg: Value=KOUTP_ACCPedalOvrd_flg_ovrdflg
      link override Signal_Override/_ovrdval: Value=KOUTP_ACCPedalOvrd_flg_ovrdval
  VVMC_ACCRequiredAccel_mps2_Inproc : FVT_lib/outp/OverrideAndLimit  SystemSampleTime=-1  VariantActivationTime=update diagram  Latency=0  AutoFrameSizeCalculation=off
      link override Signal_Limit/_maxval: Value=KOUTP_ACCRequiredAccel_mps2_maxval
      link override Signal_Limit/_minval: Value=KOUTP_ACCRequiredAccel_mps2_minval
      link override Signal_Override/_ovrdflg: Value=KOUTP_ACCRequiredAccel_mps2_ovrdflg
      link override Signal_Override/_ovrdval: Value=KOUTP_ACCRequiredAccel_mps2_ovrdval
  VVMC_ACCTakeoverReq_flg_Inproc : FVT_lib/outp/OverrideAndLimit  SystemSampleTime=-1  VariantActivationTime=update diagram  Latency=0  AutoFrameSizeCalculation=off
      link override Signal_Limit/_maxval: Value=KOUTP_ACCTakeoverReq_flg_maxval
      link override Signal_Limit/_minval: Value=KOUTP_ACCTakeoverReq_flg_minval
      link override Signal_Override/_ovrdflg: Value=KOUTP_ACCTakeoverReq_flg_ovrdflg
      link override Signal_Override/_ovrdval: Value=KOUTP_ACCTakeoverReq_flg_ovrdval
  VVMC_ACCVehHoldReq_flg_Inproc : FVT_lib/outp/OverrideAndLimit  SystemSampleTime=-1  VariantActivationTime=update diagram  Latency=0  AutoFrameSizeCalculation=off
      link override Signal_Limit/_maxval: Value=KOUTP_ACCVehHoldReq_flg_maxval
      link override Signal_Limit/_minval: Value=KOUTP_ACCVehHoldReq_flg_minval
      link override Signal_Override/_ovrdflg: Value=KOUTP_ACCVehHoldReq_flg_ovrdflg
      link override Signal_Override/_ovrdval: Value=KOUTP_ACCVehHoldReq_flg_ovrdval
  VVMC_ADASACCSta_enum_Inproc : FVT_lib/outp/OverrideAndLimit  SystemSampleTime=-1  VariantActivationTime=update diagram  Latency=0  AutoFrameSizeCalculation=off
      link override Signal_Limit/_maxval: Value=KOUTP_ADASACCSta_enum_maxval
      link override Signal_Limit/_minval: Value=KOUTP_ADASACCSta_enum_minval
      link override Signal_Override/_ovrdflg: Value=KOUTP_ADASACCSta_enum_ovrdflg
      link override Signal_Override/_ovrdval: Value=KOUTP_ADASACCSta_enum_ovrdval
  VVMC_ADASAEBReq_enum_Inproc : FVT_lib/outp/OverrideAndLimit  SystemSampleTime=-1  VariantActivationTime=update diagram  Latency=0  AutoFrameSizeCalculation=off
      link override Signal_Limit/_maxval: Value=KOUTP_ADASAEBReq_enum_maxval
      link override Signal_Limit/_minval: Value=KOUTP_ADASAEBReq_enum_minval
      link override Signal_Override/_ovrdflg: Value=KOUTP_ADASAEBReq_enum_ovrdflg
      link override Signal_Override/_ovrdval: Value=KOUTP_ADASAEBReq_enum_ovrdval
  VVMC_ADASAEBSta_enum_Inproc : FVT_lib/outp/OverrideAndLimit  SystemSampleTime=-1  VariantActivationTime=update diagram  Latency=0  AutoFrameSizeCalculation=off
      link override Signal_Limit/_maxval: Value=KOUTP_ADASAEBSta_enum_maxval
      link override Signal_Limit/_minval: Value=KOUTP_ADASAEBSta_enum_minval
      link override Signal_Override/_ovrdflg: Value=KOUTP_ADASAEBSta_enum_ovrdflg
      link override Signal_Override/_ovrdval: Value=KOUTP_ADASAEBSta_enum_ovrdval
  VVMC_ADASCAMSpdLim_enum_Inproc : FVT_lib/outp/OverrideAndLimit  SystemSampleTime=-1  VariantActivationTime=update diagram  Latency=0  AutoFrameSizeCalculation=off
      link override Signal_Limit/_maxval: Value=KOUTP_ADASCAMSpdLim_enum_maxval
      link override Signal_Limit/_minval: Value=KOUTP_ADASCAMSpdLim_enum_minval
      link override Signal_Override/_ovrdflg: Value=KOUTP_ADASCAMSpdLim_enum_ovrdflg
      link override Signal_Override/_ovrdval: Value=KOUTP_ADASCAMSpdLim_enum_ovrdval
  VVMC_ADASDBSReq_enum_Inproc : FVT_lib/outp/OverrideAndLimit  SystemSampleTime=-1  VariantActivationTime=update diagram  Latency=0  AutoFrameSizeCalculation=off
      link override Signal_Limit/_maxval: Value=KOUTP_ADASDBSReq_enum_maxval
      link override Signal_Limit/_minval: Value=KOUTP_ADASDBSReq_enum_minval
      link override Signal_Override/_ovrdflg: Value=KOUTP_ADASDBSReq_enum_ovrdflg
      link override Signal_Override/_ovrdval: Value=KOUTP_ADASDBSReq_enum_ovrdval
  VVMC_ADASFCWMute_flg_Inproc : FVT_lib/outp/OverrideAndLimit  SystemSampleTime=-1  VariantActivationTime=update diagram  Latency=0  AutoFrameSizeCalculation=off
      link override Signal_Limit/_maxval: Value=KOUTP_ADASFCWMute_flg_maxval
      link override Signal_Limit/_minval: Value=KOUTP_ADASFCWMute_flg_minval
      link override Signal_Override/_ovrdflg: Value=KOUTP_ADASFCWMute_flg_ovrdflg
      link override Signal_Override/_ovrdval: Value=KOUTP_ADASFCWMute_flg_ovrdval
  VVMC_ADASFCWSta_enum_Inproc : FVT_lib/outp/OverrideAndLimit  SystemSampleTime=-1  VariantActivationTime=update diagram  Latency=0  AutoFrameSizeCalculation=off
      link override Signal_Limit/_maxval: Value=KOUTP_ADASFCWSta_enum_maxval
      link override Signal_Limit/_minval: Value=KOUTP_ADASFCWSta_enum_minval
      link override Signal_Override/_ovrdflg: Value=KOUTP_ADASFCWSta_enum_ovrdflg
      link override Signal_Override/_ovrdval: Value=KOUTP_ADASFCWSta_enum_ovrdval
  VVMC_ADASFaultSta_flg_Inproc : FVT_lib/outp/OverrideAndLimit  SystemSampleTime=-1  VariantActivationTime=update diagram  Latency=0  AutoFrameSizeCalculation=off
      link override Signal_Limit/_maxval: Value=KOUTP_ADASFaultSta_flg_maxval
      link override Signal_Limit/_minval: Value=KOUTP_ADASFaultSta_flg_minval
      link override Signal_Override/_ovrdflg: Value=KOUTP_ADASFaultSta_flg_ovrdflg
      link override Signal_Override/_ovrdval: Value=KOUTP_ADASFaultSta_flg_ovrdval
  VVMC_ADASFltWrnReq_flg_Inproc : FVT_lib/outp/OverrideAndLimit  SystemSampleTime=-1  VariantActivationTime=update diagram  Latency=0  AutoFrameSizeCalculation=off
      link override Signal_Limit/_maxval: Value=KOUTP_ADASFltWrnReq_flg_maxval
      link override Signal_Limit/_minval: Value=KOUTP_ADASFltWrnReq_flg_minval
      link override Signal_Override/_ovrdflg: Value=KOUTP_ADASFltWrnReq_flg_ovrdflg
      link override Signal_Override/_ovrdval: Value=KOUTP_ADASFltWrnReq_flg_ovrdval
  VVMC_ADASForceIdle_flg_Inproc : FVT_lib/outp/OverrideAndLimit  SystemSampleTime=-1  VariantActivationTime=update diagram  Latency=0  AutoFrameSizeCalculation=off
      link override Signal_Limit/_maxval: Value=KOUTP_ADASForceIdle_flg_maxval
      link override Signal_Limit/_minval: Value=KOUTP_ADASForceIdle_flg_minval
      link override Signal_Override/_ovrdflg: Value=KOUTP_ADASForceIdle_flg_ovrdflg
      link override Signal_Override/_ovrdval: Value=KOUTP_ADASForceIdle_flg_ovrdval
  VVMC_ADASISASta_enum_Inproc : FVT_lib/outp/OverrideAndLimit  SystemSampleTime=-1  VariantActivationTime=update diagram  Latency=0  AutoFrameSizeCalculation=off
      link override Signal_Limit/_maxval: Value=KOUTP_ADASISASta_enum_maxval
      link override Signal_Limit/_minval: Value=KOUTP_ADASISASta_enum_minval
      link override Signal_Override/_ovrdflg: Value=KOUTP_ADASISASta_enum_ovrdflg
      link override Signal_Override/_ovrdval: Value=KOUTP_ADASISASta_enum_ovrdval
  VVMC_ADASLDWMute_flg_Inproc : FVT_lib/outp/OverrideAndLimit  SystemSampleTime=-1  VariantActivationTime=update diagram  Latency=0  AutoFrameSizeCalculation=off
      link override Signal_Limit/_maxval: Value=KOUTP_ADASLDWMute_flg_maxval
      link override Signal_Limit/_minval: Value=KOUTP_ADASLDWMute_flg_minval
      link override Signal_Override/_ovrdflg: Value=KOUTP_ADASLDWMute_flg_ovrdflg
      link override Signal_Override/_ovrdval: Value=KOUTP_ADASLDWMute_flg_ovrdval
  VVMC_ADASLDWSta_enum_Inproc : FVT_lib/outp/OverrideAndLimit  SystemSampleTime=-1  VariantActivationTime=update diagram  Latency=0  AutoFrameSizeCalculation=off
      link override Signal_Limit/_maxval: Value=KOUTP_ADASLDWSta_enum_maxval
      link override Signal_Limit/_minval: Value=KOUTP_ADASLDWSta_enum_minval
      link override Signal_Override/_ovrdflg: Value=KOUTP_ADASLDWSta_enum_ovrdflg
      link override Signal_Override/_ovrdval: Value=KOUTP_ADASLDWSta_enum_ovrdval
  VVMC_ADASLFCHandsOffWarning_enum_Inproc : FVT_lib/outp/OverrideAndLimit  SystemSampleTime=-1  VariantActivationTime=update diagram  Latency=0  AutoFrameSizeCalculation=off
      link override Signal_Limit/_maxval: Value=KOUTP_ADASLFCHandsOffWarning_enum_maxval
      link override Signal_Limit/_minval: Value=KOUTP_ADASLFCHandsOffWarning_enum_minval
      link override Signal_Override/_ovrdflg: Value=KOUTP_ADASLFCHandsOffWarning_enum_ovrdflg
      link override Signal_Override/_ovrdval: Value=KOUTP_ADASLFCHandsOffWarning_enum_ovrdval
  VVMC_ADASLFCSta_enum_Inproc : FVT_lib/outp/OverrideAndLimit  SystemSampleTime=-1  VariantActivationTime=update diagram  Latency=0  AutoFrameSizeCalculation=off
      link override Signal_Limit/_maxval: Value=KOUTP_ADASLFCSta_enum_maxval
      link override Signal_Limit/_minval: Value=KOUTP_ADASLFCSta_enum_minval
      link override Signal_Override/_ovrdflg: Value=KOUTP_ADASLFCSta_enum_ovrdflg
      link override Signal_Override/_ovrdval: Value=KOUTP_ADASLFCSta_enum_ovrdval
  VVMC_ADASLFCWarnSound_enum_Inproc : FVT_lib/outp/OverrideAndLimit  SystemSampleTime=-1  VariantActivationTime=update diagram  Latency=0  AutoFrameSizeCalculation=off
      link override Signal_Limit/_maxval: Value=KOUTP_ADASLFCWarnSound_enum_maxval
      link override Signal_Limit/_minval: Value=KOUTP_ADASLFCWarnSound_enum_minval
      link override Signal_Override/_ovrdflg: Value=KOUTP_ADASLFCWarnSound_enum_ovrdflg
      link override Signal_Override/_ovrdval: Value=KOUTP_ADASLFCWarnSound_enum_ovrdval
  VVMC_ADASLKASta_enum_Inproc : FVT_lib/outp/OverrideAndLimit  SystemSampleTime=-1  VariantActivationTime=update diagram  Latency=0  AutoFrameSizeCalculation=off
      link override Signal_Limit/_maxval: Value=KOUTP_ADASLKASta_enum_maxval
      link override Signal_Limit/_minval: Value=KOUTP_ADASLKASta_enum_minval
      link override Signal_Override/_ovrdflg: Value=KOUTP_ADASLKASta_enum_ovrdflg
      link override Signal_Override/_ovrdval: Value=KOUTP_ADASLKASta_enum_ovrdval
  VVMC_ADASLaneModeL_enum_Inproc : FVT_lib/outp/OverrideAndLimit  SystemSampleTime=-1  VariantActivationTime=update diagram  Latency=0  AutoFrameSizeCalculation=off
      link override Signal_Limit/_maxval: Value=KOUTP_ADASLaneModeL_enum_maxval
      link override Signal_Limit/_minval: Value=KOUTP_ADASLaneModeL_enum_minval
      link override Signal_Override/_ovrdflg: Value=KOUTP_ADASLaneModeL_enum_ovrdflg
      link override Signal_Override/_ovrdval: Value=KOUTP_ADASLaneModeL_enum_ovrdval
  VVMC_ADASLaneModeR_enum_Inproc : FVT_lib/outp/OverrideAndLimit  SystemSampleTime=-1  VariantActivationTime=update diagram  Latency=0  AutoFrameSizeCalculation=off
      link override Signal_Limit/_maxval: Value=KOUTP_ADASLaneModeR_enum_maxval
      link override Signal_Limit/_minval: Value=KOUTP_ADASLaneModeR_enum_minval
      link override Signal_Override/_ovrdflg: Value=KOUTP_ADASLaneModeR_enum_ovrdflg
      link override Signal_Override/_ovrdval: Value=KOUTP_ADASLaneModeR_enum_ovrdval
  VVMC_ADASLanecurveL_raw32_Inproc : FVT_lib/outp/OverrideAndLimit  SystemSampleTime=-1  VariantActivationTime=update diagram  Latency=0  AutoFrameSizeCalculation=off
      link override Signal_Limit/_maxval: Value=KOUTP_ADASLanecurveL_raw32_maxval
      link override Signal_Limit/_minval: Value=KOUTP_ADASLanecurveL_raw32_minval
      link override Signal_Override/_ovrdflg: Value=KOUTP_ADASLanecurveL_raw32_ovrdflg
      link override Signal_Override/_ovrdval: Value=KOUTP_ADASLanecurveL_raw32_ovrdval
  VVMC_ADASLanecurveR_raw32_Inproc : FVT_lib/outp/OverrideAndLimit  SystemSampleTime=-1  VariantActivationTime=update diagram  Latency=0  AutoFrameSizeCalculation=off
      link override Signal_Limit/_maxval: Value=KOUTP_ADASLanecurveR_raw32_maxval
      link override Signal_Limit/_minval: Value=KOUTP_ADASLanecurveR_raw32_minval
      link override Signal_Override/_ovrdflg: Value=KOUTP_ADASLanecurveR_raw32_ovrdflg
      link override Signal_Override/_ovrdval: Value=KOUTP_ADASLanecurveR_raw32_ovrdval
  VVMC_ADASLanetypeL_enum_Inproc : FVT_lib/outp/OverrideAndLimit  SystemSampleTime=-1  VariantActivationTime=update diagram  Latency=0  AutoFrameSizeCalculation=off
      link override Signal_Limit/_maxval: Value=KOUTP_ADASLanetypeL_enum_maxval
      link override Signal_Limit/_minval: Value=KOUTP_ADASLanetypeL_enum_minval
      link override Signal_Override/_ovrdflg: Value=KOUTP_ADASLanetypeL_enum_ovrdflg
      link override Signal_Override/_ovrdval: Value=KOUTP_ADASLanetypeL_enum_ovrdval
  VVMC_ADASLanetypeR_enum_Inproc : FVT_lib/outp/OverrideAndLimit  SystemSampleTime=-1  VariantActivationTime=update diagram  Latency=0  AutoFrameSizeCalculation=off
      link override Signal_Limit/_maxval: Value=KOUTP_ADASLanetypeR_enum_maxval
      link override Signal_Limit/_minval: Value=KOUTP_ADASLanetypeR_enum_minval
      link override Signal_Override/_ovrdflg: Value=KOUTP_ADASLanetypeR_enum_ovrdflg
      link override Signal_Override/_ovrdval: Value=KOUTP_ADASLanetypeR_enum_ovrdval
  VVMC_ADASSLIFSpdLim_enum_Inproc : FVT_lib/outp/OverrideAndLimit  SystemSampleTime=-1  VariantActivationTime=update diagram  Latency=0  AutoFrameSizeCalculation=off
      link override Signal_Limit/_maxval: Value=KOUTP_ADASSLIFSpdLim_enum_maxval
      link override Signal_Limit/_minval: Value=KOUTP_ADASSLIFSpdLim_enum_minval
      link override Signal_Override/_ovrdflg: Value=KOUTP_ADASSLIFSpdLim_enum_ovrdflg
      link override Signal_Override/_ovrdval: Value=KOUTP_ADASSLIFSpdLim_enum_ovrdval
  VVMC_ADASSLIFSta_enum_Inproc : FVT_lib/outp/OverrideAndLimit  SystemSampleTime=-1  VariantActivationTime=update diagram  Latency=0  AutoFrameSizeCalculation=off
      link override Signal_Limit/_maxval: Value=KOUTP_ADASSLIFSta_enum_maxval
      link override Signal_Limit/_minval: Value=KOUTP_ADASSLIFSta_enum_minval
      link override Signal_Override/_ovrdflg: Value=KOUTP_ADASSLIFSta_enum_ovrdflg
      link override Signal_Override/_ovrdval: Value=KOUTP_ADASSLIFSta_enum_ovrdval
  VVMC_ADASShftPosnReqA_flg_Inproc : FVT_lib/outp/OverrideAndLimit  SystemSampleTime=-1  VariantActivationTime=update diagram  Latency=0  AutoFrameSizeCalculation=off
      link override Signal_Limit/_maxval: Value=KOUTP_ADASShftPosnReqA_flg_maxval
      link override Signal_Limit/_minval: Value=KOUTP_ADASShftPosnReqA_flg_minval
      link override Signal_Override/_ovrdflg: Value=KOUTP_ADASShftPosnReqA_flg_ovrdflg
      link override Signal_Override/_ovrdval: Value=KOUTP_ADASShftPosnReqA_flg_ovrdval
  VVMC_ADASShftPosnReq_enum_Inproc : FVT_lib/outp/OverrideAndLimit  SystemSampleTime=-1  VariantActivationTime=update diagram  Latency=0  AutoFrameSizeCalculation=off
      link override Signal_Limit/_maxval: Value=KOUTP_ADASShftPosnReq_enum_maxval
      link override Signal_Limit/_minval: Value=KOUTP_ADASShftPosnReq_enum_minval
      link override Signal_Override/_ovrdflg: Value=KOUTP_ADASShftPosnReq_enum_ovrdflg
      link override Signal_Override/_ovrdval: Value=KOUTP_ADASShftPosnReq_enum_ovrdval
  VVMC_ADASVehSpdLim_raw32_Inproc : FVT_lib/outp/OverrideAndLimit  SystemSampleTime=-1  VariantActivationTime=update diagram  Latency=0  AutoFrameSizeCalculation=off
      link override Signal_Limit/_maxval: Value=KOUTP_ADASVehSpdLim_raw32_maxval
      link override Signal_Limit/_minval: Value=KOUTP_ADASVehSpdLim_raw32_minval
      link override Signal_Override/_ovrdflg: Value=KOUTP_ADASVehSpdLim_raw32_ovrdflg
      link override Signal_Override/_ovrdval: Value=KOUTP_ADASVehSpdLim_raw32_ovrdval
  VVMC_ADASWarningMsg_enum_Inproc : FVT_lib/outp/OverrideAndLimit  SystemSampleTime=-1  VariantActivationTime=update diagram  Latency=0  AutoFrameSizeCalculation=off
      link override Signal_Limit/_maxval: Value=KOUTP_ADASWarningMsg_enum_maxval
      link override Signal_Limit/_minval: Value=KOUTP_ADASWarningMsg_enum_minval
      link override Signal_Override/_ovrdflg: Value=KOUTP_ADASWarningMsg_enum_ovrdflg
      link override Signal_Override/_ovrdval: Value=KOUTP_ADASWarningMsg_enum_ovrdval
  VVMC_AEBVehHoldReq_flg_Inproc : FVT_lib/outp/OverrideAndLimit  SystemSampleTime=-1  VariantActivationTime=update diagram  Latency=0  AutoFrameSizeCalculation=off
      link override Signal_Limit/_maxval: Value=KOUTP_AEBVehHoldReq_flg_maxval
      link override Signal_Limit/_minval: Value=KOUTP_AEBVehHoldReq_flg_minval
      link override Signal_Override/_ovrdflg: Value=KOUTP_AEBVehHoldReq_flg_ovrdflg
      link override Signal_Override/_ovrdval: Value=KOUTP_AEBVehHoldReq_flg_ovrdval
  VVMC_APSActive_flg_Inproc : FVT_lib/outp/OverrideAndLimit  SystemSampleTime=-1  VariantActivationTime=update diagram  Latency=0  AutoFrameSizeCalculation=off
      link override Signal_Limit/_maxval: Value=KOUTP_APSActive_flg_maxval
      link override Signal_Limit/_minval: Value=KOUTP_APSActive_flg_minval
      link override Signal_Override/_ovrdflg: Value=KOUTP_APSActive_flg_ovrdflg
      link override Signal_Override/_ovrdval: Value=KOUTP_APSActive_flg_ovrdval
  VVMC_APSCtrlAvail_flg_Inproc : FVT_lib/outp/OverrideAndLimit  SystemSampleTime=-1  VariantActivationTime=update diagram  Latency=0  AutoFrameSizeCalculation=off
      link override Signal_Limit/_maxval: Value=KOUTP_APSCtrlAvail_flg_maxval
      link override Signal_Limit/_minval: Value=KOUTP_APSCtrlAvail_flg_minval
      link override Signal_Override/_ovrdflg: Value=KOUTP_APSCtrlAvail_flg_ovrdflg
      link override Signal_Override/_ovrdval: Value=KOUTP_APSCtrlAvail_flg_ovrdval
  VVMC_APSDecReqA_flg_Inproc : FVT_lib/outp/OverrideAndLimit  SystemSampleTime=-1  VariantActivationTime=update diagram  Latency=0  AutoFrameSizeCalculation=off
      link override Signal_Limit/_maxval: Value=KOUTP_APSDecReqA_flg_maxval
      link override Signal_Limit/_minval: Value=KOUTP_APSDecReqA_flg_minval
      link override Signal_Override/_ovrdflg: Value=KOUTP_APSDecReqA_flg_ovrdflg
      link override Signal_Override/_ovrdval: Value=KOUTP_APSDecReqA_flg_ovrdval
  VVMC_APSDecReq_mps2_Inproc : FVT_lib/outp/OverrideAndLimit  SystemSampleTime=-1  VariantActivationTime=update diagram  Latency=0  AutoFrameSizeCalculation=off
      link override Signal_Limit/_maxval: Value=KOUTP_APSDecReq_mps2_maxval
      link override Signal_Limit/_minval: Value=KOUTP_APSDecReq_mps2_minval
      link override Signal_Override/_ovrdflg: Value=KOUTP_APSDecReq_mps2_ovrdflg
      link override Signal_Override/_ovrdval: Value=KOUTP_APSDecReq_mps2_ovrdval
  VVMC_APSReq_enum_Inproc : FVT_lib/outp/OverrideAndLimit  SystemSampleTime=-1  VariantActivationTime=update diagram  Latency=0  AutoFrameSizeCalculation=off
      link override Signal_Limit/_maxval: Value=KOUTP_APSReq_enum_maxval
      link override Signal_Limit/_minval: Value=KOUTP_APSReq_enum_minval
      link override Signal_Override/_ovrdflg: Value=KOUTP_APSReq_enum_ovrdflg
      link override Signal_Override/_ovrdval: Value=KOUTP_APSReq_enum_ovrdval
  VVMC_APSStaSys_enum_Inproc : FVT_lib/outp/OverrideAndLimit  SystemSampleTime=-1  VariantActivationTime=update diagram  Latency=0  AutoFrameSizeCalculation=off
      link override Signal_Limit/_maxval: Value=KOUTP_APSStaSys_enum_maxval
      link override Signal_Limit/_minval: Value=KOUTP_APSStaSys_enum_minval
      link override Signal_Override/_ovrdflg: Value=KOUTP_APSStaSys_enum_ovrdflg
      link override Signal_Override/_ovrdval: Value=KOUTP_APSStaSys_enum_ovrdval
  VVMC_AccCalcuPID_mps2_Inproc : FVT_lib/outp/OverrideAndLimit  SystemSampleTime=-1  VariantActivationTime=update diagram  Latency=0  AutoFrameSizeCalculation=off
      link override Signal_Limit/_maxval: Value=KOUTP_AccCalcuPID_mps2_maxval
      link override Signal_Limit/_minval: Value=KOUTP_AccCalcuPID_mps2_minval
      link override Signal_Override/_ovrdflg: Value=KOUTP_AccCalcuPID_mps2_ovrdflg
      link override Signal_Override/_ovrdval: Value=KOUTP_AccCalcuPID_mps2_ovrdval
  VVMC_ActACCRequiredAccel_mps2_Inproc : FVT_lib/outp/OverrideAndLimit  SystemSampleTime=-1  VariantActivationTime=update diagram  Latency=0  AutoFrameSizeCalculation=off
      link override Signal_Limit/_maxval: Value=KOUTP_ActACCRequiredAccel_mps2_maxval
      link override Signal_Limit/_minval: Value=KOUTP_ActACCRequiredAccel_mps2_minval
      link override Signal_Override/_ovrdflg: Value=KOUTP_ActACCRequiredAccel_mps2_ovrdflg
      link override Signal_Override/_ovrdval: Value=KOUTP_ActACCRequiredAccel_mps2_ovrdval
  VVMC_CAASActive_flg_Inproc : FVT_lib/outp/OverrideAndLimit  SystemSampleTime=-1  VariantActivationTime=update diagram  Latency=0  AutoFrameSizeCalculation=off
      link override Signal_Limit/_maxval: Value=KOUTP_CAASActive_flg_maxval
      link override Signal_Limit/_minval: Value=KOUTP_CAASActive_flg_minval
      link override Signal_Override/_ovrdflg: Value=KOUTP_CAASActive_flg_ovrdflg
      link override Signal_Override/_ovrdval: Value=KOUTP_CAASActive_flg_ovrdval
  VVMC_CAASCtrlAvail_flg_Inproc : FVT_lib/outp/OverrideAndLimit  SystemSampleTime=-1  VariantActivationTime=update diagram  Latency=0  AutoFrameSizeCalculation=off
      link override Signal_Limit/_maxval: Value=KOUTP_CAASCtrlAvail_flg_maxval
      link override Signal_Limit/_minval: Value=KOUTP_CAASCtrlAvail_flg_minval
      link override Signal_Override/_ovrdflg: Value=KOUTP_CAASCtrlAvail_flg_ovrdflg
      link override Signal_Override/_ovrdval: Value=KOUTP_CAASCtrlAvail_flg_ovrdval
  VVMC_CCCtrlSta_enum_Inproc : FVT_lib/outp/OverrideAndLimit  SystemSampleTime=-1  VariantActivationTime=update diagram  Latency=0  AutoFrameSizeCalculation=off
      link override Signal_Limit/_maxval: Value=KOUTP_CCCtrlSta_enum_maxval
      link override Signal_Limit/_minval: Value=KOUTP_CCCtrlSta_enum_minval
      link override Signal_Override/_ovrdflg: Value=KOUTP_CCCtrlSta_enum_ovrdflg
      link override Signal_Override/_ovrdval: Value=KOUTP_CCCtrlSta_enum_ovrdval
  VVMC_CCMSASpdWar_flg_Inproc : FVT_lib/outp/OverrideAndLimit  SystemSampleTime=-1  VariantActivationTime=update diagram  Latency=0  AutoFrameSizeCalculation=off
      link override Signal_Limit/_maxval: Value=KOUTP_CCMSASpdWar_flg_maxval
      link override Signal_Limit/_minval: Value=KOUTP_CCMSASpdWar_flg_minval
      link override Signal_Override/_ovrdflg: Value=KOUTP_CCMSASpdWar_flg_ovrdflg
      link override Signal_Override/_ovrdval: Value=KOUTP_CCMSASpdWar_flg_ovrdval
  VVMC_CalibratedAccX_G_Inproc : FVT_lib/outp/OverrideAndLimit  SystemSampleTime=-1  VariantActivationTime=update diagram  Latency=0  AutoFrameSizeCalculation=off
